simulink model "ICAC_AutoSave_20200630_1355"  (R2018b)
settings: Solver=FixedStepDiscrete  StartTime=0.0  StopTime=10.0  RelTol=1e-3
InitFcn:
  | tmpVer = ver('MATLAB');
  | tmpVer = str2num(tmpVer.Version);
  | % -------------------------------------------------------------------
  | %  MATLAB file generated by Simulink.saveVars on 21-Nov-2019 10:06:14
  | %  MATLAB version: 7.13.0.564 (R2011b)
  | % -------------------------------------------------------------------
  | 
  | 
  | SInt16 = Simulink.AliasType;
  | SInt16.Description = 'Num';
  | if (tmpVer > 7.11)
  | 	SInt16.DataScope = 'Auto';
  | end
  | SInt16.HeaderFile = 'Rte_Type.h';
  | SInt16.BaseType = 'int16';
  | 
  | SInt32 = Simulink.AliasType;
  | SInt32.Description = 'Num';
  | if (tmpVer > 7.11)
  | 	SInt32.DataScope = 'Auto';
  | end
  | SInt32.HeaderFile = 'Rte_Type.h';
  | SInt32.BaseType = 'int32';
  | 
  | SInt8 = Simulink.AliasType;
  | SInt8.Description = 'Num';
  | if (tmpVer > 7.11)
  | 	SInt8.DataScope = 'Auto';
  | end
  | SInt8.HeaderFile = 'Rte_Type.h';
  | SInt8.BaseType = 'int8';
  | 
  | T_A_m2_1024_1_u32 = Simulink.NumericType;
  | T_A_m2_1024_1_u32.Description = 'm2 (square meters  (m2))';
  | if (tmpVer > 7.11)
  | 	T_A_m2_1024_1_u32.DataScope = 'Auto';
  | end
  | T_A_m2_1024_1_u32.HeaderFile = 'Rte_Type.h';
  | T_A_m2_1024_1_u32.DataTypeMode = 'Fixed-point: slope and bias scaling';
  | T_A_m2_1024_1_u32.SignednessBool = false;
  | T_A_m2_1024_1_u32.WordLength = 32;
  | T_A_m2_1024_1_u32.FixedExponent = -10;
  | T_A_m2_1024_1_u32.SlopeAdjustmentFactor = 1;
  | T_A_m2_1024_1_u32.Bias = 0;
  | T_A_m2_1024_1_u32.DataTypeOverride = 'Inherit';
  | T_A_m2_1024_1_u32.IsAlias = true;
  | 
  | T_A_m2_65536_1_u16 = Simulink.NumericType;
  | T_A_m2_65536_1_u16.Description = 'm2 (square meters  (m2))';
  | if (tmpVer > 7.11)
  | 	T_A_m2_65536_1_u16.DataScope = 'Auto';
  | end
  | T_A_m2_65536_1_u16.HeaderFile = 'Rte_Type.h';
  | T_A_m2_65536_1_u16.DataTypeMode = 'Fixed-point: slope and bias scaling';
  | T_A_m2_65536_1_u16.SignednessBool = false;
  | T_A_m2_65536_1_u16.WordLength = 16;
  | T_A_m2_65536_1_u16.FixedExponent = -16;
  | T_A_m2_65536_1_u16.SlopeAdjustmentFactor = 1;
  | T_A_m2_65536_1_u16.Bias = 0;
  | T_A_m2_65536_1_u16.DataTypeOverride = 'Inherit';
  | ... (+4598 lines)
StopFcn:
  | clear  T_A_m2_1024_1_u32 T_A_m2_65536_1_u16 T_A_m2_Float32 T_A_mm2_10_1_u16 T_A_mm2_4_1_s16 T_A_mm2_Float32 T_Cnt_Num_10_1_u32 T_Cnt_Num_1_1_s16 T_Cnt_Num_1_1_s32 T_Cnt_Num_1_1_s8 T_Cnt_Num_1_1_u16 T_Cnt_Num_1_1_u32 T_Cnt_Num_1_1_u8 T_E_J_1_1_s32 T_E_J_Float32 T_E_kJ_128_1_s32 T_E_kJ_Float32 T_E_kwh_10_1_u16 T_E_kwh_Float32 T_Epl_kwhpkm_100_1_u16 T_Epl_kwhpkm_Float32 T_F_N_1_1_s16 T_F_N_Float32 T_I_A_1000_1_u16 T_I_A_1048576_1_s32 T_I_A_2048_1_s16 T_I_A_32_1_s16 T_I_A_Float32 T_I_mA_1_1_s16 T_I_mA_32768_128_s16 T_I_mA_Float32 T_J_kgpm2_128_1_u16 T_J_kgpm2_Float32 T_K_NA_1000_1_s16 T_K_NA_100_1_s16 T_K_NA_100_1_u16 T_K_NA_1024_1_s16 T_K_NA_1024_1_u16 T_K_NA_128_1_s16 T_K_NA_128_1_u16 T_K_NA_128_1_u8 T_K_NA_16777216_1_u32 T_K_NA_16_1_s16 T_K_NA_16_1_u16 T_K_NA_16_1_u8 T_K_NA_1_16_u16 T_K_NA_1_1_s16 T_K_NA_1_1_u16 T_K_NA_1_1_u8 T_K_NA_32768_1_s16 T_K_NA_32768_1_u16 T_K_NA_32_1_s8 T_K_NA_4096_1_u16 T_K_NA_4194304_1_s32 T_K_NA_4194304_1_u16 T_K_NA_65536_1_s32 T_K_NA_65536_1_u16 T_K_NA_8192_1_s16 T_K_NA_8_1_s16 T_K_NA_Float32 T_M_Nm_16_1_s16 T_M_Nm_1_1_s16 T_M_Nm_32768_1_s16 T_M_Nm_32_1_s16 T_M_Nm_4_1_s16 T_M_Nm_512_1_s16 T_M_Nm_Float32 T_P_W_1_4_s16 T_P_W_1_8_s16 T_P_W_Float32 T_P_kW_128_1_s16 T_P_kW_1_8_s16 T_P_kW_8_1_s32 T_P_kW_Float32 T_Pct_pct_1024_1_s32 T_Pct_pct_1024_1_u32 T_Pct_pct_10_1_s16 T_Pct_pct_10_1_u32 T_Pct_pct_128_100_s8 T_Pct_pct_1_1_s16 T_Pct_pct_1_4_u8 T_Pct_pct_255_100_u16 T_Pct_pct_255_100_u8 T_Pct_pct_256_1_s16 T_Pct_pct_256_1_u16 T_Pct_pct_65535_100_u16 T_Pct_pct_Float32 T_R_ohm_1024_1_s16 T_R_ohm_32_1_s16 T_R_ohm_Float32 T_TK_K_16_1_s16 T_TK_K_Float32 T_T_degC_10_400_1_u16 T_T_degC_16_1_s16 T_T_degC_1_40_1_u8 T_T_degC_2_80_1_u8 T_T_degC_Float32 T_U_V_1000_1_u16 T_U_V_10_1_u8 T_U_V_200_1_u8 T_U_V_32_1_s16 T_U_V_4096_1_s16 T_U_V_512_1_s16 T_U_V_65535_8_u16 T_U_V_8192_1_u16 T_U_V_Float32 T_U_mV_1_1_s16 T_U_mV_256_20_u16 T_U_mV_Float32 T_V_l_256_1_s16 T_V_l_4096_1_s16 T_V_l_64_1_s16 T_V_l_65535_100_u16 T_V_l_Float32 T_V_ml_128_1_s16 T_V_ml_1_1_s16 T_V_ml_32768_1_s16 T_V_ml_Float32 T_V_ul_32_1_u16 T_V_ul_Float32 T_Vpl_clpkm_512_1_u16 T_Vpl_clpkm_Float32 T_a_kphps_16_1_s16 T_a_kphps_Float32 T_a_mps2_128_1_s16 T_a_mps2_Float32 T_c_MJpkg_256_1_s16 T_c_MJpkg_Float32 T_c_kJpgpK_1024_1_s16 T_c_kJpgpK_Float32 T_c_kJpkgpK_128_1_u16 T_c_kJpkgpK_Float32 T_chrg_Ah_1_1_s16 T_chrg_Ah_1_1_u16 T_chrg_Ah_1_1_u8 T_chrg_Ah_256_1_u16 T_chrg_Ah_4194304_1_s32 T_chrg_Ah_512_1_u16 T_chrg_Ah_8_1_u16 T_chrg_Ah_Float32 T_cmp_NA_100_1_s16 T_cmp_NA_128_1_s16 T_cmp_NA_16_1_s16 T_cmp_NA_32768_1_u16 T_cmp_NA_Float32 T_d2n_rpmps2_4_1_s16 T_d2n_rpmps2_Float32 T_dPct_pctps_16_1_s16 T_dPct_pctps_256_1_s16 T_dPct_pctps_Float32 T_dT_degCps_128_1_s16 T_dT_degCps_Float32 T_dV_lph_1_1_s16 T_dV_lph_Float32 T_dV_lpm_128_1_s16 T_dV_lpm_32_1_s16 T_dV_lpm_Float32 T_dV_lps_1024_1_u16 T_dV_lps_4_1_u16 T_dV_lps_Float32 T_dV_mlps_1024_1_s16 T_dV_mlps_Float32 T_d_BitField16 T_dm_gps_128_1_s16 T_dm_gps_128_1_u16 T_dm_gps_256_1_u16 T_dm_gps_Float32 T_dm_mgps_1_1_s16 T_dm_mgps_Float32 T_dn_rpmps_1_1_s16 T_dn_rpmps_2_1_s16 T_dn_rpmps_Float32 T_dp_Paps_1_1_s16 T_dp_Paps_Float32 T_dp_kPaps_1_1_s16 T_dp_kPaps_8_1_s16 T_dp_kPaps_Float32 T_dphi_degps_128_1_s16 T_dphi_degps_8_1_s16 T_dphi_degps_Float32 T_dr_ps_256_1_s16 T_dr_ps_Float32 T_drho_mgplps_1_2_s16 T_drho_mgplps_Float32 T_e_NA_1_1_u8 T_f_Hz_1_1_u16 T_f_Hz_1_1_u32 T_f_Hz_64_1_u16 T_f_Hz_8_1_s16 T_f_Hz_Float32 T_g_BitField32 T_l_km_16_1_s16 T_l_km_1_1_u16 T_l_km_1_1_u32 T_l_km_Float32 T_l_m_1024_1_s16 T_l_m_16_1_s16 T_l_m_1_1_u32 T_l_m_Float32 T_l_mm_16_1_s16 T_l_mm_1_1_u16 T_l_mm_4096_1_s16 T_l_mm_4_1_u8 T_l_mm_64_1_s16 T_l_mm_Float32 T_m_g_1_1_s16 T_m_g_2048_1_s16 T_m_g_32_1_u16 T_m_g_Float32 T_m_kg_1024_1_s16 T_m_kg_1_1_s16 T_m_kg_1_1_u32 T_m_kg_Float32 T_m_mg_128_1_s16 T_m_mg_32_1_s16 T_m_mg_Float32 T_n_rpm_1_1_s16 T_n_rpm_1_25_u8 T_n_rpm_256_50_u16 T_n_rpm_2_25_u8 T_n_rpm_4_1_u16 T_n_rpm_Float32 T_p_MPa_64_1_s16 T_p_MPa_Float32 T_p_Pa_1_1_s16 T_p_Pa_Float32 T_p_kPa_1_10_u16 T_p_kPa_1_1_s16 T_p_kPa_1_1_u8 T_p_kPa_256_1_u16 T_p_kPa_32_1_u16 T_p_kPa_64_1_s16 T_p_kPa_Float32 T_phi_deg_100_1_s16 T_phi_deg_1024_1_s16 T_phi_deg_128_1_s16 T_phi_deg_1_1_u8 T_phi_deg_256_1_s16 T_phi_deg_2_1_s8 T_phi_deg_32_1_s16 T_phi_deg_512_6_s32 T_phi_deg_Float32 T_phi_rad_2048_1_s16 T_phi_rad_Float32 T_r_NA_1024_1_s16 T_r_NA_1024_1_u16 T_r_NA_16384_1_s16 T_r_NA_16_1_s16 T_r_NA_256_1_s8 T_r_NA_256_1_u16 T_r_NA_32768_1_u16 T_r_NA_32_1_u16 T_r_NA_4096_1_s16 T_r_NA_65535_2_u16 T_r_NA_8192_1_u16 T_r_NA_Float32 T_rho_gpl_8192_1_s16 T_rho_gpl_Float32 T_rho_kgpm3_16_1_s16 T_rho_kgpm3_Float32 T_rho_mgpl_1_1_s16 T_rho_mgpl_64_1_s16 T_rho_mgpl_Float32 T_t_hour_1_1_s16 T_t_hour_Float32 T_t_m_1_1_u16 T_t_m_Float32 T_t_ms_1_1_s16 T_t_ms_1_1_u16 T_t_ms_1_1_u32 T_t_ms_4096_1_s16 T_t_ms_64_1_s16 T_t_ms_Float32 T_t_s_1000_1_s16 T_t_s_100_1_s16 T_t_s_10_1_s16 T_t_s_10_1_u16 T_t_s_1_1_s16 T_t_s_1_1_u16 T_t_s_1_1_u32 T_t_s_Float32 T_t_us_10_1_u32 T_t_us_1_1_s16 T_t_us_1_1_u32 T_t_us_1_4_u16 T_t_us_Float32 T_v_kph_1_1_u8 T_v_kph_64_1_s16 T_v_kph_64_1_u16 T_v_kph_Float32 T_v_mps_256_1_s16 T_v_mps_Float32 T_w_radps_32_1_s16 T_w_radps_Float32 T_y_BitField8 T_y_BitFieldDiagProgress T_y_BitFieldDiagStatus T_y_NA_1_1_u8 SInt16 SInt32 SInt8 T_BOOLEAN UInt16 UInt32 UInt8 s16 s32 s8 u16 u32 u8
(part 3 of 3)

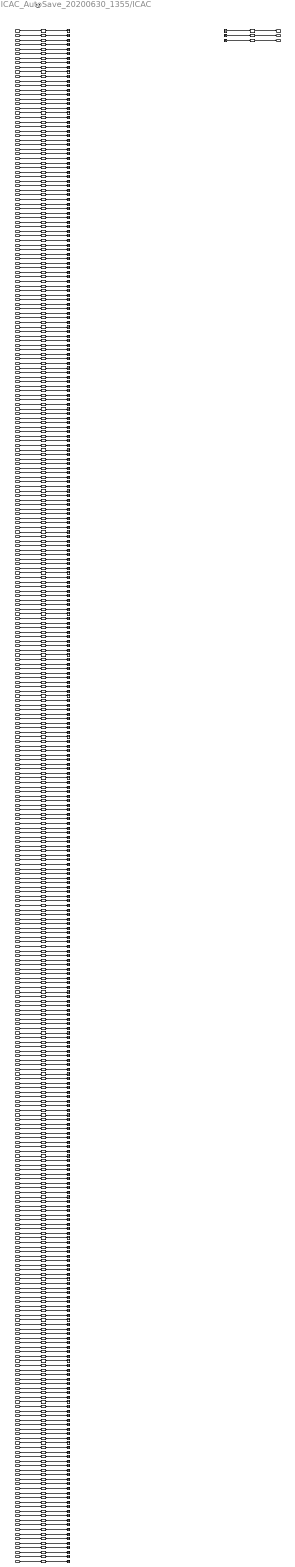
== system ICAC_AutoSave_20200630_1355/ICAC ==
  System_Clock : Inport
  ICABva_g_VehParameter : Inport  Port=2
  ICABva_g_FilterInfo : Inport  Port=3
  ICABve_d_SignalTStamp : Inport  Port=4
  ICAPva_g_PathPoints : Inport  Port=5
  ICAPve_d_PathPointNum : Inport  Port=6
  ICAPve_d_PathValid : Inport  Port=7
  ICAPve_d_SignalTStamp : Inport  Port=8
  ICASva_g_TrajectoryPoints : Inport  Port=9
  ICASve_d_TrajectoryPointNum : Inport  Port=10
  ICASve_d_TrajectoryValid : Inport  Port=11
  ICASva_d_TrajectoryPlanState : Inport  Port=12
  ICASve_g_ExpLonAcc : Inport  Port=13
  ICASve_d_SignalTStamp : Inport  Port=14
  IMAPve_d_EPS_LKA_State : Inport  Port=15
  IMAPve_g_EPS_SW_Trq : Inport  Port=16
  IMAPve_d_EPS_Error_State : Inport  Port=17
  IMAPve_d_EPS_Trq_State : Inport  Port=18
  IMAPve_d_SAS_Clb_State : Inport  Port=19
  IMAPve_d_SAS_Trim_State : Inport  Port=20
  IMAPve_d_EPS_TrqLim_State : Inport  Port=21
  IMAPve_g_EPS_LKA_Current : Inport  Port=22
  IMAPve_g_ESC_LatAcc : Inport  Port=23
  IMAPve_d_ESC_LatAcc_Valid : Inport  Port=24
  IMAPve_g_ESC_YawRate : Inport  Port=25
  IMAPve_d_ESC_YawRate_Valid : Inport  Port=26
  IMAPve_g_ESC_UnYawRate : Inport  Port=27
  IMAPve_g_ESC_VehSpd : Inport  Port=28
  IMAPve_g_ESC_LonAcc : Inport  Port=29
  IMAPve_d_ESC_LonAcc_Valid : Inport  Port=30
  IMAPve_g_ESC_Brake_Press : Inport  Port=31
  IMAPve_g_ESC_Static_Slope : Inport  Port=32
  IMAPve_g_ESC_DySlope_Accuracy : Inport  Port=33
  IMAPve_g_ESC_DySlope : Inport  Port=34
  IMAPve_g_SW_Angle : Inport  Port=35
  IMAPve_g_SW_Angle_Speed : Inport  Port=36
  IMAPve_d_BCM_HazardLamp : Inport  Port=37
  IMAPve_d_BCM_Left_Light : Inport  Port=38
  IMAPve_d_BCM_Right_Light : Inport  Port=39
  IMAPve_d_ESC_BrakeLamp_Req : Inport  Port=40
  IMAPve_d_BCM_Opening_State : Inport  Port=41
  IMAPve_d_BCM_Trunk_State : Inport  Port=42
  IMAPve_d_BCM_LF_Door_State : Inport  Port=43
  IMAPve_d_BCM_RF_Door_State : Inport  Port=44
  IMAPve_d_BCM_RR_Door_State : Inport  Port=45
  IMAPve_d_BCM_LR_Door_State : Inport  Port=46
  IMAPve_d_SCC_Left_SwitchSig : Inport  Port=47
  IMAPve_d_SCC_Right_SwitchSig : Inport  Port=48
  IMAPve_d_PEPS_Door_Lock_Req : Inport  Port=49
  IMAPve_d_BCM_Door_Lock_State : Inport  Port=50
  IMAPve_d_EMS_ACC_Status : Inport  Port=51
  IMAPve_g_EMS_Pot_WhlT_Max : Inport  Port=52
  IMAPve_g_EMS_Pot_WhlT_Min : Inport  Port=53
  IMAPve_g_EMS_RealPedal : Inport  Port=54
  IMAPve_g_EMS_MaxTWhl : Inport  Port=55
  IMAPve_g_EMS_MaxTWhl_Offset : Inport  Port=56
  IMAPve_g_EMS_MinTWhl : Inport  Port=57
  IMAPve_g_EMS_MinTWhl_Offset : Inport  Port=58
  IMAPve_g_EMS_Actual_FlwT : Inport  Port=59
  IMAPve_g_EMS_Actual_IndT : Inport  Port=60
  IMAPve_g_EMS_Realize_TWhl : Inport  Port=61
  IMAPve_g_EMS_ACC_VirtualPedal : Inport  Port=62
  IMAPve_d_EMS_AccPedal_Fault : Inport  Port=63
  IMAPve_g_EMS_Driver_Torque : Inport  Port=64
  IMAPve_d_ESC_Brake_Effort : Inport  Port=65
  IMAPve_g_EMS_Engine_Speed : Inport  Port=66
  IMAPve_d_ESC_Veh_Standstill : Inport  Port=67
  IMAPve_d_TCU_Actual_Gear : Inport  Port=68
  IMAPve_d_TCU_Target_Gear : Inport  Port=69
  IMAPve_d_TCU_PRND_State : Inport  Port=70
  IMAPve_d_BCM_Ignition_State : Inport  Port=71
  IMAPve_d_ACU_Driver_Belt : Inport  Port=72
  IMAPve_d_SWS_Fault_Code : Inport  Port=73
  IMAPve_d_SWS_Failure_Status : Inport  Port=74
  IMAPve_d_ESC_OFF : Inport  Port=75
  IMAPve_d_ESC_AlarmSig : Inport  Port=76
  IMAPve_d_Speed_Limit_Switch : Inport  Port=77
  IMAPve_d_ESC_ESC_Active : Inport  Port=78
  IMAPve_d_ESC_MSR_Active : Inport  Port=79
  IMAPve_d_ESC_TCS_Active : Inport  Port=80
  IMAPve_d_ESC_VehSpd_Valid : Inport  Port=81
  IMAPve_d_Brake_Pedal_Fault : Inport  Port=82
  IMAPve_d_ESC_ABS_Active : Inport  Port=83
  IMAPve_d_ESC_ABS_Valid : Inport  Port=84
  IMAPve_d_ESC_ABS_AlarmSig : Inport  Port=85
  IMAPve_d_ESC_FL_WheelPulVal : Inport  Port=86
  IMAPve_d_ESC_FR_WheelPulVal : Inport  Port=87
  IMAPve_d_ESC_RL_WheelPulVal : Inport  Port=88
  IMAPve_d_ESC_RR_WheelPulVal : Inport  Port=89
  IMAPve_g_ESC_FL_WhlSpd : Inport  Port=90
  IMAPve_d_ESC_FL_WhlSpd_Fault : Inport  Port=91
  IMAPve_g_ESC_FR_WhlSpd : Inport  Port=92
  IMAPve_d_ESC_FR_WhlSpd_Fault : Inport  Port=93
  IMAPve_g_ESC_RL_WhlSpd : Inport  Port=94
  IMAPve_d_ESC_RL_WhlSpd_Fault : Inport  Port=95
  IMAPve_g_ESC_RR_WhlSpd : Inport  Port=96
  IMAPve_d_ESC_RR_WhlSpd_Fault : Inport  Port=97
  IMAPve_d_ESC_FL_Wheel_Pulse : Inport  Port=98
  IMAPve_d_ESC_FR_Wheel_Pulse : Inport  Port=99
  IMAPve_d_ESC_RL_Wheel_Pulse : Inport  Port=100
  IMAPve_d_ESC_RR_Wheel_Pulse : Inport  Port=101
  IMAPve_d_TCU_AT_Failure : Inport  Port=102
  IMAPve_d_TCU_Shift_Valid : Inport  Port=103
  IMAPve_d_TCU_DCT_Clutch_State : Inport  Port=104
  IMAPve_d_TCU_Gear_Engage : Inport  Port=105
  IMAPve_d_TCU_Select_ATMode : Inport  Port=106
  IMAPve_d_EMS_Engine_Status : Inport  Port=107
  IMAPve_d_EMS_Gearbox_CtlAvail : Inport  Port=108
  IMAPve_d_ESC_Brake_Failsafe : Inport  Port=109
  IMAPve_d_ESC_AEB_Status : Inport  Port=110
  IMAPve_d_ESC_AEB_Available : Inport  Port=111
  IMAPve_d_ESC_AEB_Active : Inport  Port=112
  IMAPve_d_ESC_ACC_Status : Inport  Port=113
  IMAPve_d_ESC_ACC_Available : Inport  Port=114
  IMAPve_d_ESC_ACC_Active : Inport  Port=115
  IMAPve_d_EMS_ACC_Effective : Inport  Port=116
  IMAPve_d_BCM_FrontWiper_State : Inport  Port=117
  IMAPve_d_BCM_CHMSL_Status : Inport  Port=118
  IMAPve_d_BCM_BrakeLamp_State : Inport  Port=119
  IMAPve_d_GW_Brake_Only_Req : Inport  Port=120
  IMAPve_d_ACU_Passenger_Belt : Inport  Port=121
  IMAPve_d_EMS_ACC_CtlAvail : Inport  Port=122
  IMAPve_d_EMS_ACC_Inhibited : Inport  Port=123
  IMAPve_d_EMS_Brake_Pedal : Inport  Port=124
  IMAPve_d_BCM_LowBeam_State : Inport  Port=125
  IMAPve_d_BCM_HighBeam_State : Inport  Port=126
  IMAPve_d_EPB_Status : Inport  Port=127
  IMAPve_d_EPB_Display_Req : Inport  Port=128
  IMAPve_d_EPB_Warn_Req : Inport  Port=129
  IMAPve_d_EPB_Switch_State : Inport  Port=130
  IMAPve_d_EPB_Switch_Valid : Inport  Port=131
  IMAPve_d_ESC_Drive_Direction : Inport  Port=132
  IMAPve_d_ESC_Hold_State : Inport  Port=133
  IMAPve_d_EPS_Steer_Hold_State : Inport  Port=134
  IMAPve_d_EPS_Warning_State : Inport  Port=135
  IMAPve_g_EPS_PowerCon : Inport  Port=136
  IMAPve_d_ESC_EBD_AlarmSig : Inport  Port=137
  IMAPve_d_ESC_AVH_Status : Inport  Port=138
  IMAPve_d_Radar_Detective_Req : Inport  Port=139
  IMAPve_g_BCM_Battery_Voltage : Inport  Port=140
  IMAPve_d_TBOX_LocalTimeY : Inport  Port=141
  IMAPve_d_TBOX_LocalTimeM : Inport  Port=142
  IMAPve_d_TBOX_LocalTimeD : Inport  Port=143
  IMAPve_d_TBOX_LocalTimeH : Inport  Port=144
  IMAPve_d_TBOX_LocalTimeMin : Inport  Port=145
  IMAPve_d_TBOX_LocalTimeS : Inport  Port=146
  IMAPve_d_TBOX_LocalTime_Valid : Inport  Port=147
  IMAPve_d_TPMS_Warn_Indicate : Inport  Port=148
  IMAPve_d_Radar_State : Inport  Port=149
  IMAPve_d_ACC_Desired_Headway : Inport  Port=150
  IMAPve_d_Time_System_Clock : Inport  Port=151
  IMAPve_d_Signal_Time_Stamp : Inport  Port=152
  IMAPve_g_GW_IC_Odometer : Inport  Port=153
  IMAPve_g_FAPA_State : Inport  Port=154
  IMAPve_d_Outside_Temp : Inport  Port=155
  IMAPve_d_ORI_CIPV_ID : Inport  Port=156
  IMAPve_d_ORI_Obj_Num : Inport  Port=157
  IMAPva_g_ORI_Probability : Inport  Port=158
  IMAPva_d_ORI_Obj_Class : Inport  Port=159
  IMAPva_d_ORI_Obj_Motion : Inport  Port=160
  IMAPva_g_ORI_Obj_RelVel : Inport  Port=161
  IMAPva_g_ORI_Obj_LongDis : Inport  Port=162
  IMAPva_d_ORI_Obj_Lane : Inport  Port=163
  IMAPva_g_ORI_Obj_LAngle : Inport  Port=164
  IMAPva_g_ORI_Obj_RAngle : Inport  Port=165
  IMAPva_g_ORI_Obj_Width : Inport  Port=166
  IMAPva_d_ORI_Obj_ID : Inport  Port=167
  IMAPve_d_ORI_Lane_Valid : Inport  Port=168
  IMAPve_d_ORI_Lane_ConsArea : Inport  Port=169
  IMAPve_d_ORI_Lane_RoadType : Inport  Port=170
  IMAPve_g_ORI_L0_C3 : Inport  Port=171
  IMAPve_g_ORI_L0_C2 : Inport  Port=172
  IMAPve_g_ORI_L0_C1 : Inport  Port=173
  IMAPve_g_ORI_L0_C0 : Inport  Port=174
  IMAPve_d_ORI_L0_Q : Inport  Port=175
  IMAPve_d_ORI_L0_Type : Inport  Port=176
  IMAPve_g_ORI_L0_VR : Inport  Port=177
  IMAPve_g_ORI_L0_TLC : Inport  Port=178
  IMAPve_g_ORI_L0_W : Inport  Port=179
  IMAPve_d_ORI_L0_LC : Inport  Port=180
  IMAPve_g_ORI_L1_C3 : Inport  Port=181
  IMAPve_g_ORI_L1_C2 : Inport  Port=182
  IMAPve_g_ORI_L1_C1 : Inport  Port=183
  IMAPve_g_ORI_L1_C0 : Inport  Port=184
  IMAPve_d_ORI_L1_Q : Inport  Port=185
  IMAPve_d_ORI_L1_Type : Inport  Port=186
  IMAPve_g_ORI_L1_VR : Inport  Port=187
  IMAPve_g_ORI_L1_TLC : Inport  Port=188
  IMAPve_g_ORI_L1_W : Inport  Port=189
  IMAPve_d_ORI_L1_LC : Inport  Port=190
  IMAPve_g_ORI_R0_C3 : Inport  Port=191
  IMAPve_g_ORI_R0_C2 : Inport  Port=192
  IMAPve_g_ORI_R0_C1 : Inport  Port=193
  IMAPve_g_ORI_R0_C0 : Inport  Port=194
  IMAPve_d_ORI_R0_Q : Inport  Port=195
  IMAPve_d_ORI_R0_LT : Inport  Port=196
  IMAPve_g_ORI_R0_VR : Inport  Port=197
  IMAPve_g_ORI_R0_TLC : Inport  Port=198
  IMAPve_g_ORI_R0_W : Inport  Port=199
  IMAPve_d_ORI_R0_LC : Inport  Port=200
  IMAPve_g_ORI_R1_C3 : Inport  Port=201
  IMAPve_g_ORI_R1_C2 : Inport  Port=202
  IMAPve_g_ORI_R1_C1 : Inport  Port=203
  IMAPve_g_ORI_R1_C0 : Inport  Port=204
  IMAPve_d_ORI_R1_Q : Inport  Port=205
  IMAPve_d_ORI_R1_LT : Inport  Port=206
  IMAPve_g_ORI_R1_VR : Inport  Port=207
  IMAPve_g_ORI_R1_TLC : Inport  Port=208
  IMAPve_g_ORI_R1_W : Inport  Port=209
  IMAPve_d_ORI_R1_LC : Inport  Port=210
  IMAPve_d_Sensor_Status : Inport  Port=211
  IMAPve_d_LF_Radar_Status : Inport  Port=212
  IMAPve_d_RF_Radar_Status : Inport  Port=213
  IMAPve_d_LR_Radar_Status : Inport  Port=214
  IMAPve_d_RR_Radar_Status : Inport  Port=215
  IMAPve_d_Fusion_Status : Inport  Port=216
  IMAPve_g_Fusion_Time_Stamp : Inport  Port=217
  IMAPve_d_obj_Num : Inport  Port=218
  IMAPva_d_obj_id : Inport  Port=219
  IMAPva_g_obj_pos_x : Inport  Port=220
  IMAPva_g_obj_pos_y : Inport  Port=221
  IMAPva_g_obj_vel_x : Inport  Port=222
  IMAPva_g_obj_vel_y : Inport  Port=223
  IMAPva_g_obj_acc_x : Inport  Port=224
  IMAPva_g_obj_acc_y : Inport  Port=225
  IMAPva_g_obj_pos_var_x : Inport  Port=226
  IMAPva_g_obj_pos_var_y : Inport  Port=227
  IMAPva_g_obj_pos_var_xy : Inport  Port=228
  IMAPva_g_obj_vel_var_x : Inport  Port=229
  IMAPva_g_obj_vel_var_y : Inport  Port=230
  IMAPva_g_obj_vel_var_xy : Inport  Port=231
  IMAPva_g_obj_width : Inport  Port=232
  IMAPva_g_obj_length : Inport  Port=233
  IMAPva_d_obj_fusion_type : Inport  Port=234
  IMAPva_d_obj_class : Inport  Port=235
  IMAPva_d_obj_lane : Inport  Port=236
  IMAPva_d_obj_status : Inport  Port=237
  IMAPva_d_obj_cam_asso_id : Inport  Port=238
  IMAPva_g_obj_con : Inport  Port=239
  IMAPva_g_obj_age : Inport  Port=240
  IMAPva_d_obj_TurnLight : Inport  Port=241
  IMAPva_d_obj_BrakeLight : Inport  Port=242
  IMAPva_d_obj_MotionStatus : Inport  Port=243
  IMAPva_d_obj_ACC : Inport  Port=244
  IMAPva_d_obj_AEB : Inport  Port=245
  IMAPva_d_obj_ELK : Inport  Port=246
  IMAPva_d_obj_ALC : Inport  Port=247
  IMAPva_d_obj_ESA : Inport  Port=248
  IMAPva_d_obj_JA : Inport  Port=249
  IMAPve_d_Lane_Valid : Inport  Port=250
  IMAPve_d_Road_Type : Inport  Port=251
  IMAPve_d_ConsArea : Inport  Port=252
  IMAPve_g_L0_C0 : Inport  Port=253
  IMAPve_g_L0_C1 : Inport  Port=254
  IMAPve_g_L0_C2 : Inport  Port=255
  IMAPve_g_L0_C3 : Inport  Port=256
  IMAPve_g_L0_VR : Inport  Port=257
  IMAPve_d_L0_Q : Inport  Port=258
  IMAPve_d_L0_Type : Inport  Port=259
  IMAPve_g_L0_Confidence : Inport  Port=260
  IMAPve_g_L0_W : Inport  Port=261
  IMAPve_g_L0_TLC : Inport  Port=262
  IMAPve_d_L0_LC : Inport  Port=263
  IMAPve_g_R0_C0 : Inport  Port=264
  IMAPve_g_R0_C1 : Inport  Port=265
  IMAPve_g_R0_C2 : Inport  Port=266
  IMAPve_g_R0_C3 : Inport  Port=267
  IMAPve_g_R0_VR : Inport  Port=268
  IMAPve_d_R0_Q : Inport  Port=269
  IMAPve_d_R0_Type : Inport  Port=270
  IMAPve_g_R0_Confidence : Inport  Port=271
  IMAPve_g_R0_W : Inport  Port=272
  IMAPve_g_R0_TLC : Inport  Port=273
  IMAPve_d_R0_LC : Inport  Port=274
  IMAPve_g_L1_C0 : Inport  Port=275
  IMAPve_g_L1_C1 : Inport  Port=276
  IMAPve_g_L1_C2 : Inport  Port=277
  IMAPve_g_L1_C3 : Inport  Port=278
  IMAPve_g_L1_VR : Inport  Port=279
  IMAPve_d_L1_Q : Inport  Port=280
  IMAPve_d_L1_Type : Inport  Port=281
  IMAPve_g_L1_Confidence : Inport  Port=282
  IMAPve_g_L1_W : Inport  Port=283
  IMAPve_g_L1_TLC : Inport  Port=284
  IMAPve_d_L1_LC : Inport  Port=285
  IMAPve_g_R1_C0 : Inport  Port=286
  IMAPve_g_R1_C1 : Inport  Port=287
  IMAPve_g_R1_C2 : Inport  Port=288
  IMAPve_g_R1_C3 : Inport  Port=289
  IMAPve_g_R1_VR : Inport  Port=290
  IMAPve_d_R1_Q : Inport  Port=291
  IMAPve_d_R1_Type : Inport  Port=292
  IMAPve_g_R1_Confidence : Inport  Port=293
  IMAPve_g_R1_W : Inport  Port=294
  IMAPve_g_R1_TLC : Inport  Port=295
  IMAPve_d_R1_LC : Inport  Port=296
  IMAPve_g_L0_C0_Back : Inport  Port=297
  IMAPve_g_L0_C1_Back : Inport  Port=298
  IMAPve_g_L0_C2_Back : Inport  Port=299
  IMAPve_g_L0_C3_Back : Inport  Port=300
  IMAPve_g_L0_Range_Back : Inport  Port=301
  IMAPve_g_L0_C0_FR_Pred : Inport  Port=302
  IMAPve_g_L0_C1_FR_Pred : Inport  Port=303
  IMAPve_g_L0_C2_FR_Pred : Inport  Port=304
  IMAPve_g_L0_Range_FR_Pred : Inport  Port=305
  IMAPve_g_R0_C0_Back : Inport  Port=306
  IMAPve_g_R0_C1_Back : Inport  Port=307
  IMAPve_g_R0_C2_Back : Inport  Port=308
  IMAPve_g_R0_C3_Back : Inport  Port=309
  IMAPve_g_R0_Range_Back : Inport  Port=310
  IMAPve_g_R0_C0_FR_Pred : Inport  Port=311
  IMAPve_g_R0_C1_FR_Pred : Inport  Port=312
  IMAPve_g_R0_C2_FR_Pred : Inport  Port=313
  IMAPve_g_R0_Range_FR_Pred : Inport  Port=314
  IMAPve_g_L1_C0_Back : Inport  Port=315
  IMAPve_g_L1_C1_Back : Inport  Port=316
  IMAPve_g_L1_C2_Back : Inport  Port=317
  IMAPve_g_L1_C3_Back : Inport  Port=318
  IMAPve_g_L1_Range_Back : Inport  Port=319
  IMAPve_g_L1_C0_FR_Pred : Inport  Port=320
  IMAPve_g_L1_C1_FR_Pred : Inport  Port=321
  IMAPve_g_L1_C2_FR_Pred : Inport  Port=322
  IMAPve_g_L1_Range_FR_Pred : Inport  Port=323
  IMAPve_g_R1_C0_Back : Inport  Port=324
  IMAPve_g_R1_C1_Back : Inport  Port=325
  IMAPve_g_R1_C2_Back : Inport  Port=326
  IMAPve_g_R1_C3_Back : Inport  Port=327
  IMAPve_g_R1_Range_Back : Inport  Port=328
  IMAPve_g_R1_C0_FR_Pred : Inport  Port=329
  IMAPve_g_R1_C1_FR_Pred : Inport  Port=330
  IMAPve_g_R1_C2_FR_Pred : Inport  Port=331
  IMAPve_g_R1_Range_FR_Pred : Inport  Port=332
  IMAPve_d_Sign_ISA_Value : Inport  Port=333
  IMAPve_d_TSR_Sign_Type : Inport  Port=334
  IMAPve_d_Camera_Signal_Fault : Inport  Port=335
  IMAPve_d_Radar_Status : Inport  Port=336
  IMAPve_d_Camera_Status : Inport  Port=337
  function : TriggerPort  TriggerType=function-call  VariantControl=Variant  SampleTimeType=periodic  SampleTime=-1
  ICABva_g_FilterInfo_1 : DataTypeConversion  OutDataTypeStr=single
  ICABva_g_FilterInfo_2 : Terminator
  ICABva_g_VehParameter1 : Terminator
  ICABva_g_VehParameter_1 : DataTypeConversion  OutDataTypeStr=single
  ICABve_d_SignalTStamp_1 : DataTypeConversion  OutDataTypeStr=uint16
  ICABve_d_SignalTStamp_2 : Terminator
  ICACve_d_SignalTStamp_1 : DataTypeConversion  OutDataTypeStr=UInt16
  ICACve_d_SignalTStamp_2 : Ground
  ICACve_d_SteerAngleVld_1 : DataTypeConversion  OutDataTypeStr=UInt16
  ICACve_d_SteerAngleVld_2 : Ground
  ICACve_g_SteerAngleCmd_1 : DataTypeConversion  OutDataTypeStr=T_M_Nm_Float32
  ICACve_g_SteerAngleCmd_2 : Ground
  ICAPva_g_PathPoints_1 : DataTypeConversion  OutDataTypeStr=single
  ICAPva_g_PathPoints_2 : Terminator
  ICAPve_d_PathPointNum_1 : DataTypeConversion  OutDataTypeStr=uint16
  ICAPve_d_PathPointNum_2 : Terminator
  ICAPve_d_PathValid_1 : DataTypeConversion  OutDataTypeStr=uint16
  ICAPve_d_PathValid_2 : Terminator
  ICAPve_d_SignalTStamp_1 : DataTypeConversion  OutDataTypeStr=uint16
  ICAPve_d_SignalTStamp_2 : Terminator
  ICASva_d_TrajectoryPlanState_1 : DataTypeConversion  OutDataTypeStr=uint16
  ICASva_d_TrajectoryPlanState_2 : Terminator
  ICASva_g_TrajectoryPoints_1 : DataTypeConversion  OutDataTypeStr=single
  ICASva_g_TrajectoryPoints_2 : Terminator
  ICASve_d_SignalTStamp_1 : DataTypeConversion  OutDataTypeStr=uint16
  ICASve_d_SignalTStamp_2 : Terminator
  ICASve_d_TrajectoryPointNum_1 : DataTypeConversion  OutDataTypeStr=uint16
  ICASve_d_TrajectoryPointNum_2 : Terminator
  ICASve_d_TrajectoryValid_1 : DataTypeConversion  OutDataTypeStr=uint16
  ICASve_d_TrajectoryValid_2 : Terminator
  ICASve_g_ExpLonAcc_1 : DataTypeConversion  OutDataTypeStr=single
  ICASve_g_ExpLonAcc_2 : Terminator
  IMAPva_d_ORI_Obj_Class_1 : DataTypeConversion  OutDataTypeStr=uint16
  IMAPva_d_ORI_Obj_Class_2 : Terminator
  IMAPva_d_ORI_Obj_ID_1 : DataTypeConversion  OutDataTypeStr=uint16
  IMAPva_d_ORI_Obj_ID_2 : Terminator
  IMAPva_d_ORI_Obj_Lane_1 : DataTypeConversion  OutDataTypeStr=uint16
  IMAPva_d_ORI_Obj_Lane_2 : Terminator
  IMAPva_d_ORI_Obj_Motion_1 : DataTypeConversion  OutDataTypeStr=uint16
  IMAPva_d_ORI_Obj_Motion_2 : Terminator
  IMAPva_d_obj_ACC_1 : DataTypeConversion  OutDataTypeStr=uint16
  IMAPva_d_obj_ACC_2 : Terminator
  IMAPva_d_obj_AEB_1 : DataTypeConversion  OutDataTypeStr=uint16
  IMAPva_d_obj_AEB_2 : Terminator
  IMAPva_d_obj_ALC_1 : DataTypeConversion  OutDataTypeStr=uint16
  IMAPva_d_obj_ALC_2 : Terminator
  IMAPva_d_obj_BrakeLight_1 : DataTypeConversion  OutDataTypeStr=uint16
  IMAPva_d_obj_BrakeLight_2 : Terminator
  IMAPva_d_obj_ELK_1 : DataTypeConversion  OutDataTypeStr=uint16
  IMAPva_d_obj_ELK_2 : Terminator
  IMAPva_d_obj_ESA_1 : DataTypeConversion  OutDataTypeStr=uint16
  IMAPva_d_obj_ESA_2 : Terminator
  IMAPva_d_obj_JA_1 : DataTypeConversion  OutDataTypeStr=uint16
  IMAPva_d_obj_JA_2 : Terminator
  IMAPva_d_obj_MotionStatus_1 : DataTypeConversion  OutDataTypeStr=uint16
  IMAPva_d_obj_MotionStatus_2 : Terminator
  IMAPva_d_obj_TurnLight_1 : DataTypeConversion  OutDataTypeStr=uint16
  IMAPva_d_obj_TurnLight_2 : Terminator
  IMAPva_d_obj_cam_asso_id_1 : DataTypeConversion  OutDataTypeStr=uint16
  IMAPva_d_obj_cam_asso_id_2 : Terminator
  IMAPva_d_obj_class_1 : DataTypeConversion  OutDataTypeStr=uint16
  IMAPva_d_obj_class_2 : Terminator
  IMAPva_d_obj_fusion_type_1 : DataTypeConversion  OutDataTypeStr=uint16
  IMAPva_d_obj_fusion_type_2 : Terminator
  IMAPva_d_obj_id_1 : DataTypeConversion  OutDataTypeStr=uint16
  IMAPva_d_obj_id_2 : Terminator
  IMAPva_d_obj_lane_1 : DataTypeConversion  OutDataTypeStr=uint16
  IMAPva_d_obj_lane_2 : Terminator
  IMAPva_d_obj_status_1 : DataTypeConversion  OutDataTypeStr=uint16
  IMAPva_d_obj_status_2 : Terminator
  IMAPva_g_ORI_Obj_LAngle_1 : DataTypeConversion  OutDataTypeStr=single
  IMAPva_g_ORI_Obj_LAngle_2 : Terminator
  IMAPva_g_ORI_Obj_LongDis_1 : DataTypeConversion  OutDataTypeStr=single
  IMAPva_g_ORI_Obj_LongDis_2 : Terminator
  IMAPva_g_ORI_Obj_RAngle_1 : DataTypeConversion  OutDataTypeStr=single
  IMAPva_g_ORI_Obj_RAngle_2 : Terminator
  IMAPva_g_ORI_Obj_RelVel_1 : DataTypeConversion  OutDataTypeStr=single
  IMAPva_g_ORI_Obj_RelVel_2 : Terminator
  IMAPva_g_ORI_Obj_Width_1 : DataTypeConversion  OutDataTypeStr=single
  IMAPva_g_ORI_Obj_Width_2 : Terminator
  IMAPva_g_ORI_Probability_1 : DataTypeConversion  OutDataTypeStr=single
  IMAPva_g_ORI_Probability_2 : Terminator
  IMAPva_g_obj_acc_x_1 : DataTypeConversion  OutDataTypeStr=single
  IMAPva_g_obj_acc_x_2 : Terminator
  IMAPva_g_obj_acc_y_1 : DataTypeConversion  OutDataTypeStr=single
  IMAPva_g_obj_acc_y_2 : Terminator
  IMAPva_g_obj_age_1 : DataTypeConversion  OutDataTypeStr=single
  IMAPva_g_obj_age_2 : Terminator
  IMAPva_g_obj_con_1 : DataTypeConversion  OutDataTypeStr=single
  IMAPva_g_obj_con_2 : Terminator
  IMAPva_g_obj_length_1 : DataTypeConversion  OutDataTypeStr=single
  IMAPva_g_obj_length_2 : Terminator
  IMAPva_g_obj_pos_var_x_1 : DataTypeConversion  OutDataTypeStr=single
  IMAPva_g_obj_pos_var_x_2 : Terminator
  IMAPva_g_obj_pos_var_xy_1 : DataTypeConversion  OutDataTypeStr=single
  IMAPva_g_obj_pos_var_xy_2 : Terminator
  IMAPva_g_obj_pos_var_y_1 : DataTypeConversion  OutDataTypeStr=single
  IMAPva_g_obj_pos_var_y_2 : Terminator
  IMAPva_g_obj_pos_x_1 : DataTypeConversion  OutDataTypeStr=single
  IMAPva_g_obj_pos_x_2 : Terminator
  IMAPva_g_obj_pos_y_1 : DataTypeConversion  OutDataTypeStr=single
  IMAPva_g_obj_pos_y_2 : Terminator
  IMAPva_g_obj_vel_var_x_1 : DataTypeConversion  OutDataTypeStr=single
  IMAPva_g_obj_vel_var_x_2 : Terminator
  IMAPva_g_obj_vel_var_xy_1 : DataTypeConversion  OutDataTypeStr=single
  IMAPva_g_obj_vel_var_xy_2 : Terminator
  IMAPva_g_obj_vel_var_y_1 : DataTypeConversion  OutDataTypeStr=single
  IMAPva_g_obj_vel_var_y_2 : Terminator
  IMAPva_g_obj_vel_x_1 : DataTypeConversion  OutDataTypeStr=single
  IMAPva_g_obj_vel_x_2 : Terminator
  IMAPva_g_obj_vel_y_1 : DataTypeConversion  OutDataTypeStr=single
  IMAPva_g_obj_vel_y_2 : Terminator
  IMAPva_g_obj_width_1 : DataTypeConversion  OutDataTypeStr=single
  IMAPva_g_obj_width_2 : Terminator
  IMAPve_d_ACC_Desired_Headway_1 : DataTypeConversion  OutDataTypeStr=uint16
  IMAPve_d_ACC_Desired_Headway_2 : Terminator
  IMAPve_d_ACU_Driver_Belt_1 : DataTypeConversion  OutDataTypeStr=uint16
  IMAPve_d_ACU_Driver_Belt_2 : Terminator
  IMAPve_d_ACU_Passenger_Belt_1 : DataTypeConversion  OutDataTypeStr=uint16
  IMAPve_d_ACU_Passenger_Belt_2 : Terminator
  IMAPve_d_BCM_BrakeLamp_State_1 : DataTypeConversion  OutDataTypeStr=uint16
  IMAPve_d_BCM_BrakeLamp_State_2 : Terminator
  IMAPve_d_BCM_CHMSL_Status_1 : DataTypeConversion  OutDataTypeStr=uint16
  IMAPve_d_BCM_CHMSL_Status_2 : Terminator
  IMAPve_d_BCM_Door_Lock_State_1 : DataTypeConversion  OutDataTypeStr=uint16
  IMAPve_d_BCM_Door_Lock_State_2 : Terminator
  IMAPve_d_BCM_FrontWiper_State_1 : DataTypeConversion  OutDataTypeStr=uint16
  IMAPve_d_BCM_FrontWiper_State_2 : Terminator
  IMAPve_d_BCM_HazardLamp_1 : DataTypeConversion  OutDataTypeStr=uint16
  IMAPve_d_BCM_HazardLamp_2 : Terminator
  IMAPve_d_BCM_HighBeam_State_1 : DataTypeConversion  OutDataTypeStr=uint16
  IMAPve_d_BCM_HighBeam_State_2 : Terminator
  IMAPve_d_BCM_Ignition_State_1 : DataTypeConversion  OutDataTypeStr=uint16
  IMAPve_d_BCM_Ignition_State_2 : Terminator
  IMAPve_d_BCM_LF_Door_State_1 : DataTypeConversion  OutDataTypeStr=uint16
  IMAPve_d_BCM_LF_Door_State_2 : Terminator
  IMAPve_d_BCM_LR_Door_State_1 : DataTypeConversion  OutDataTypeStr=uint16
  IMAPve_d_BCM_LR_Door_State_2 : Terminator
  IMAPve_d_BCM_Left_Light_1 : DataTypeConversion  OutDataTypeStr=uint16
  IMAPve_d_BCM_Left_Light_2 : Terminator
  IMAPve_d_BCM_LowBeam_State_1 : DataTypeConversion  OutDataTypeStr=uint16
  IMAPve_d_BCM_LowBeam_State_2 : Terminator
  IMAPve_d_BCM_Opening_State_1 : DataTypeConversion  OutDataTypeStr=uint16
  IMAPve_d_BCM_Opening_State_2 : Terminator
  IMAPve_d_BCM_RF_Door_State_1 : DataTypeConversion  OutDataTypeStr=uint16
  IMAPve_d_BCM_RF_Door_State_2 : Terminator
  IMAPve_d_BCM_RR_Door_State_1 : DataTypeConversion  OutDataTypeStr=uint16
  IMAPve_d_BCM_RR_Door_State_2 : Terminator
  IMAPve_d_BCM_Right_Light_1 : DataTypeConversion  OutDataTypeStr=uint16
  IMAPve_d_BCM_Right_Light_2 : Terminator
  IMAPve_d_BCM_Trunk_State_1 : DataTypeConversion  OutDataTypeStr=uint16
  IMAPve_d_BCM_Trunk_State_2 : Terminator
  IMAPve_d_Brake_Pedal_Fault_1 : DataTypeConversion  OutDataTypeStr=uint16
  IMAPve_d_Brake_Pedal_Fault_2 : Terminator
  IMAPve_d_Camera_Signal_Fault_1 : DataTypeConversion  OutDataTypeStr=uint16
  IMAPve_d_Camera_Signal_Fault_2 : Terminator
  IMAPve_d_Camera_Status_1 : DataTypeConversion  OutDataTypeStr=uint16
  IMAPve_d_Camera_Status_2 : Terminator
  IMAPve_d_ConsArea_1 : DataTypeConversion  OutDataTypeStr=uint16
  IMAPve_d_ConsArea_2 : Terminator
  IMAPve_d_EMS_ACC_CtlAvail_1 : DataTypeConversion  OutDataTypeStr=uint16
  IMAPve_d_EMS_ACC_CtlAvail_2 : Terminator
  IMAPve_d_EMS_ACC_Effective_1 : DataTypeConversion  OutDataTypeStr=uint16
  IMAPve_d_EMS_ACC_Effective_2 : Terminator
  IMAPve_d_EMS_ACC_Inhibited_1 : DataTypeConversion  OutDataTypeStr=uint16
  IMAPve_d_EMS_ACC_Inhibited_2 : Terminator
  IMAPve_d_EMS_ACC_Status_1 : DataTypeConversion  OutDataTypeStr=uint16
  IMAPve_d_EMS_ACC_Status_2 : Terminator
  IMAPve_d_EMS_AccPedal_Fault_1 : DataTypeConversion  OutDataTypeStr=uint16
  IMAPve_d_EMS_AccPedal_Fault_2 : Terminator
  IMAPve_d_EMS_Brake_Pedal_1 : DataTypeConversion  OutDataTypeStr=uint16
  IMAPve_d_EMS_Brake_Pedal_2 : Terminator
  IMAPve_d_EMS_Engine_Status_1 : DataTypeConversion  OutDataTypeStr=uint16
  IMAPve_d_EMS_Engine_Status_2 : Terminator
  IMAPve_d_EMS_Gearbox_CtlAvail_1 : DataTypeConversion  OutDataTypeStr=uint16
  IMAPve_d_EMS_Gearbox_CtlAvail_2 : Terminator
  IMAPve_d_EPB_Display_Req_1 : DataTypeConversion  OutDataTypeStr=uint16
  IMAPve_d_EPB_Display_Req_2 : Terminator
  IMAPve_d_EPB_Status_1 : DataTypeConversion  OutDataTypeStr=uint16
  IMAPve_d_EPB_Status_2 : Terminator
  IMAPve_d_EPB_Switch_State_1 : DataTypeConversion  OutDataTypeStr=uint16
  IMAPve_d_EPB_Switch_State_2 : Terminator
  IMAPve_d_EPB_Switch_Valid_1 : DataTypeConversion  OutDataTypeStr=uint16
  IMAPve_d_EPB_Switch_Valid_2 : Terminator
  IMAPve_d_EPB_Warn_Req_1 : DataTypeConversion  OutDataTypeStr=uint16
  IMAPve_d_EPB_Warn_Req_2 : Terminator
  IMAPve_d_EPS_Error_State_1 : DataTypeConversion  OutDataTypeStr=uint16
  IMAPve_d_EPS_Error_State_2 : Terminator
  IMAPve_d_EPS_LKA_State_1 : DataTypeConversion  OutDataTypeStr=uint16
  IMAPve_d_EPS_LKA_State_2 : Terminator
  IMAPve_d_EPS_Steer_Hold_State_1 : DataTypeConversion  OutDataTypeStr=uint16
  IMAPve_d_EPS_Steer_Hold_State_2 : Terminator
  IMAPve_d_EPS_TrqLim_State_1 : DataTypeConversion  OutDataTypeStr=uint16
  IMAPve_d_EPS_TrqLim_State_2 : Terminator
  IMAPve_d_EPS_Trq_State_1 : DataTypeConversion  OutDataTypeStr=uint16
  IMAPve_d_EPS_Trq_State_2 : Terminator
  IMAPve_d_EPS_Warning_State_1 : DataTypeConversion  OutDataTypeStr=uint16
  IMAPve_d_EPS_Warning_State_2 : Terminator
  IMAPve_d_ESC_ABS_Active_1 : DataTypeConversion  OutDataTypeStr=uint16
  IMAPve_d_ESC_ABS_Active_2 : Terminator
  IMAPve_d_ESC_ABS_AlarmSig_1 : DataTypeConversion  OutDataTypeStr=uint16
  IMAPve_d_ESC_ABS_AlarmSig_2 : Terminator
  IMAPve_d_ESC_ABS_Valid_1 : DataTypeConversion  OutDataTypeStr=uint16
  IMAPve_d_ESC_ABS_Valid_2 : Terminator
  IMAPve_d_ESC_ACC_Active_1 : DataTypeConversion  OutDataTypeStr=uint16
  IMAPve_d_ESC_ACC_Active_2 : Terminator
  IMAPve_d_ESC_ACC_Available_1 : DataTypeConversion  OutDataTypeStr=uint16
  IMAPve_d_ESC_ACC_Available_2 : Terminator
  IMAPve_d_ESC_ACC_Status_1 : DataTypeConversion  OutDataTypeStr=uint16
  IMAPve_d_ESC_ACC_Status_2 : Terminator
  IMAPve_d_ESC_AEB_Active_1 : DataTypeConversion  OutDataTypeStr=uint16
  IMAPve_d_ESC_AEB_Active_2 : Terminator
  IMAPve_d_ESC_AEB_Available_1 : DataTypeConversion  OutDataTypeStr=uint16
  IMAPve_d_ESC_AEB_Available_2 : Terminator
  IMAPve_d_ESC_AEB_Status_1 : DataTypeConversion  OutDataTypeStr=uint16
  IMAPve_d_ESC_AEB_Status_2 : Terminator
  IMAPve_d_ESC_AVH_Status_1 : DataTypeConversion  OutDataTypeStr=uint16
  IMAPve_d_ESC_AVH_Status_2 : Terminator
  IMAPve_d_ESC_AlarmSig_1 : DataTypeConversion  OutDataTypeStr=uint16
  IMAPve_d_ESC_AlarmSig_2 : Terminator
  IMAPve_d_ESC_BrakeLamp_Req_1 : DataTypeConversion  OutDataTypeStr=uint16
  IMAPve_d_ESC_BrakeLamp_Req_2 : Terminator
  IMAPve_d_ESC_Brake_Effort_1 : DataTypeConversion  OutDataTypeStr=uint16
  IMAPve_d_ESC_Brake_Effort_2 : Terminator
  IMAPve_d_ESC_Brake_Failsafe_1 : DataTypeConversion  OutDataTypeStr=uint16
  IMAPve_d_ESC_Brake_Failsafe_2 : Terminator
  IMAPve_d_ESC_Drive_Direction_1 : DataTypeConversion  OutDataTypeStr=uint16
  IMAPve_d_ESC_Drive_Direction_2 : Terminator
  IMAPve_d_ESC_EBD_AlarmSig_1 : DataTypeConversion  OutDataTypeStr=uint16
  IMAPve_d_ESC_EBD_AlarmSig_2 : Terminator
  IMAPve_d_ESC_ESC_Active_1 : DataTypeConversion  OutDataTypeStr=uint16
  IMAPve_d_ESC_ESC_Active_2 : Terminator
  IMAPve_d_ESC_FL_WheelPulVal_1 : DataTypeConversion  OutDataTypeStr=uint16
  IMAPve_d_ESC_FL_WheelPulVal_2 : Terminator
  IMAPve_d_ESC_FL_Wheel_Pulse_1 : DataTypeConversion  OutDataTypeStr=uint16
  IMAPve_d_ESC_FL_Wheel_Pulse_2 : Terminator
  IMAPve_d_ESC_FL_WhlSpd_Fault_1 : DataTypeConversion  OutDataTypeStr=uint16
  IMAPve_d_ESC_FL_WhlSpd_Fault_2 : Terminator
  IMAPve_d_ESC_FR_WheelPulVal_1 : DataTypeConversion  OutDataTypeStr=uint16
  IMAPve_d_ESC_FR_WheelPulVal_2 : Terminator
  IMAPve_d_ESC_FR_Wheel_Pulse_1 : DataTypeConversion  OutDataTypeStr=uint16
  IMAPve_d_ESC_FR_Wheel_Pulse_2 : Terminator
  IMAPve_d_ESC_FR_WhlSpd_Fault_1 : DataTypeConversion  OutDataTypeStr=uint16
  IMAPve_d_ESC_FR_WhlSpd_Fault_2 : Terminator
  IMAPve_d_ESC_Hold_State_1 : DataTypeConversion  OutDataTypeStr=uint16
  IMAPve_d_ESC_Hold_State_2 : Terminator
  IMAPve_d_ESC_LatAcc_Valid_1 : DataTypeConversion  OutDataTypeStr=uint16
  IMAPve_d_ESC_LatAcc_Valid_2 : Terminator
  IMAPve_d_ESC_LonAcc_Valid_1 : DataTypeConversion  OutDataTypeStr=uint16
  IMAPve_d_ESC_LonAcc_Valid_2 : Terminator
  IMAPve_d_ESC_MSR_Active_1 : DataTypeConversion  OutDataTypeStr=uint16
  IMAPve_d_ESC_MSR_Active_2 : Terminator
  IMAPve_d_ESC_OFF_1 : DataTypeConversion  OutDataTypeStr=uint16
  IMAPve_d_ESC_OFF_2 : Terminator
  IMAPve_d_ESC_RL_WheelPulVal_1 : DataTypeConversion  OutDataTypeStr=uint16
  IMAPve_d_ESC_RL_WheelPulVal_2 : Terminator
  IMAPve_d_ESC_RL_Wheel_Pulse_1 : DataTypeConversion  OutDataTypeStr=uint16
  IMAPve_d_ESC_RL_Wheel_Pulse_2 : Terminator
  IMAPve_d_ESC_RL_WhlSpd_Fault_1 : DataTypeConversion  OutDataTypeStr=uint16
  IMAPve_d_ESC_RL_WhlSpd_Fault_2 : Terminator
  IMAPve_d_ESC_RR_WheelPulVal_1 : DataTypeConversion  OutDataTypeStr=uint16
  IMAPve_d_ESC_RR_WheelPulVal_2 : Terminator
  IMAPve_d_ESC_RR_Wheel_Pulse_1 : DataTypeConversion  OutDataTypeStr=uint16
  IMAPve_d_ESC_RR_Wheel_Pulse_2 : Terminator
  IMAPve_d_ESC_RR_WhlSpd_Fault_1 : DataTypeConversion  OutDataTypeStr=uint16
  IMAPve_d_ESC_RR_WhlSpd_Fault_2 : Terminator
  IMAPve_d_ESC_TCS_Active_1 : DataTypeConversion  OutDataTypeStr=uint16
  IMAPve_d_ESC_TCS_Active_2 : Terminator
  IMAPve_d_ESC_VehSpd_Valid_1 : DataTypeConversion  OutDataTypeStr=uint16
  IMAPve_d_ESC_VehSpd_Valid_2 : Terminator
  IMAPve_d_ESC_Veh_Standstill_1 : DataTypeConversion  OutDataTypeStr=uint16
  IMAPve_d_ESC_Veh_Standstill_2 : Terminator
  IMAPve_d_ESC_YawRate_Valid_1 : DataTypeConversion  OutDataTypeStr=uint16
  IMAPve_d_ESC_YawRate_Valid_2 : Terminator
  IMAPve_d_Fusion_Status_1 : DataTypeConversion  OutDataTypeStr=uint16
  IMAPve_d_Fusion_Status_2 : Terminator
  IMAPve_d_GW_Brake_Only_Req_1 : DataTypeConversion  OutDataTypeStr=uint16
  IMAPve_d_GW_Brake_Only_Req_2 : Terminator
  IMAPve_d_L0_LC_1 : DataTypeConversion  OutDataTypeStr=uint16
  IMAPve_d_L0_LC_2 : Terminator
  IMAPve_d_L0_Q_1 : DataTypeConversion  OutDataTypeStr=uint16
  IMAPve_d_L0_Q_2 : Terminator
  IMAPve_d_L0_Type_1 : DataTypeConversion  OutDataTypeStr=uint16
  IMAPve_d_L0_Type_2 : Terminator
  IMAPve_d_L1_LC_1 : DataTypeConversion  OutDataTypeStr=uint16
  IMAPve_d_L1_LC_2 : Terminator
  IMAPve_d_L1_Q_1 : DataTypeConversion  OutDataTypeStr=uint16
  IMAPve_d_L1_Q_2 : Terminator
  IMAPve_d_L1_Type_1 : DataTypeConversion  OutDataTypeStr=uint16
  IMAPve_d_L1_Type_2 : Terminator
  IMAPve_d_LF_Radar_Status_1 : DataTypeConversion  OutDataTypeStr=uint16
  IMAPve_d_LF_Radar_Status_2 : Terminator
  IMAPve_d_LR_Radar_Status_1 : DataTypeConversion  OutDataTypeStr=uint16
  IMAPve_d_LR_Radar_Status_2 : Terminator
  IMAPve_d_Lane_Valid_1 : DataTypeConversion  OutDataTypeStr=uint16
  IMAPve_d_Lane_Valid_2 : Terminator
  IMAPve_d_ORI_CIPV_ID_1 : DataTypeConversion  OutDataTypeStr=uint16
  IMAPve_d_ORI_CIPV_ID_2 : Terminator
  IMAPve_d_ORI_L0_LC_1 : DataTypeConversion  OutDataTypeStr=uint16
  IMAPve_d_ORI_L0_LC_2 : Terminator
  IMAPve_d_ORI_L0_Q_1 : DataTypeConversion  OutDataTypeStr=uint16
  IMAPve_d_ORI_L0_Q_2 : Terminator
  IMAPve_d_ORI_L0_Type_1 : DataTypeConversion  OutDataTypeStr=uint16
  IMAPve_d_ORI_L0_Type_2 : Terminator
  IMAPve_d_ORI_L1_LC_1 : DataTypeConversion  OutDataTypeStr=uint16
  IMAPve_d_ORI_L1_LC_2 : Terminator
  IMAPve_d_ORI_L1_Q_1 : DataTypeConversion  OutDataTypeStr=uint16
  IMAPve_d_ORI_L1_Q_2 : Terminator
  IMAPve_d_ORI_L1_Type_1 : DataTypeConversion  OutDataTypeStr=uint16
  IMAPve_d_ORI_L1_Type_2 : Terminator
  IMAPve_d_ORI_Lane_ConsArea_1 : DataTypeConversion  OutDataTypeStr=uint16
  IMAPve_d_ORI_Lane_ConsArea_2 : Terminator
  IMAPve_d_ORI_Lane_RoadType_1 : DataTypeConversion  OutDataTypeStr=uint16
  IMAPve_d_ORI_Lane_RoadType_2 : Terminator
  IMAPve_d_ORI_Lane_Valid_1 : DataTypeConversion  OutDataTypeStr=uint16
  IMAPve_d_ORI_Lane_Valid_2 : Terminator
  IMAPve_d_ORI_Obj_Num_1 : DataTypeConversion  OutDataTypeStr=uint16
  IMAPve_d_ORI_Obj_Num_2 : Terminator
  IMAPve_d_ORI_R0_LC_1 : DataTypeConversion  OutDataTypeStr=uint16
  IMAPve_d_ORI_R0_LC_2 : Terminator
  IMAPve_d_ORI_R0_LT_1 : DataTypeConversion  OutDataTypeStr=uint16
  IMAPve_d_ORI_R0_LT_2 : Terminator
  IMAPve_d_ORI_R0_Q_1 : DataTypeConversion  OutDataTypeStr=uint16
  IMAPve_d_ORI_R0_Q_2 : Terminator
  IMAPve_d_ORI_R1_LC_1 : DataTypeConversion  OutDataTypeStr=uint16
  IMAPve_d_ORI_R1_LC_2 : Terminator
  IMAPve_d_ORI_R1_LT_1 : DataTypeConversion  OutDataTypeStr=uint16
  IMAPve_d_ORI_R1_LT_2 : Terminator
  IMAPve_d_ORI_R1_Q_1 : DataTypeConversion  OutDataTypeStr=uint16
  IMAPve_d_ORI_R1_Q_2 : Terminator
  IMAPve_d_Outside_Temp_1 : DataTypeConversion  OutDataTypeStr=uint16
  IMAPve_d_Outside_Temp_2 : Terminator
  IMAPve_d_PEPS_Door_Lock_Req_1 : DataTypeConversion  OutDataTypeStr=uint16
  IMAPve_d_PEPS_Door_Lock_Req_2 : Terminator
  IMAPve_d_R0_LC_1 : DataTypeConversion  OutDataTypeStr=uint16
  IMAPve_d_R0_LC_2 : Terminator
  IMAPve_d_R0_Q_1 : DataTypeConversion  OutDataTypeStr=uint16
  IMAPve_d_R0_Q_2 : Terminator
  IMAPve_d_R0_Type_1 : DataTypeConversion  OutDataTypeStr=uint16
  IMAPve_d_R0_Type_2 : Terminator
  IMAPve_d_R1_LC_1 : DataTypeConversion  OutDataTypeStr=uint16
  IMAPve_d_R1_LC_2 : Terminator
  IMAPve_d_R1_Q_1 : DataTypeConversion  OutDataTypeStr=uint16
  IMAPve_d_R1_Q_2 : Terminator
  IMAPve_d_R1_Type_1 : DataTypeConversion  OutDataTypeStr=uint16
  IMAPve_d_R1_Type_2 : Terminator
  IMAPve_d_RF_Radar_Status_1 : DataTypeConversion  OutDataTypeStr=uint16
  IMAPve_d_RF_Radar_Status_2 : Terminator
  IMAPve_d_RR_Radar_Status_1 : DataTypeConversion  OutDataTypeStr=uint16
  IMAPve_d_RR_Radar_Status_2 : Terminator
  IMAPve_d_Radar_Detective_Req_1 : DataTypeConversion  OutDataTypeStr=uint16
  IMAPve_d_Radar_Detective_Req_2 : Terminator
  IMAPve_d_Radar_State_1 : DataTypeConversion  OutDataTypeStr=uint16
  IMAPve_d_Radar_State_2 : Terminator
  IMAPve_d_Radar_Status_1 : DataTypeConversion  OutDataTypeStr=uint16
  IMAPve_d_Radar_Status_2 : Terminator
  IMAPve_d_Road_Type_1 : DataTypeConversion  OutDataTypeStr=uint16
  IMAPve_d_Road_Type_2 : Terminator
  IMAPve_d_SAS_Clb_State_1 : DataTypeConversion  OutDataTypeStr=uint16
  IMAPve_d_SAS_Clb_State_2 : Terminator
  IMAPve_d_SAS_Trim_State_1 : DataTypeConversion  OutDataTypeStr=uint16
  IMAPve_d_SAS_Trim_State_2 : Terminator
  IMAPve_d_SCC_Left_SwitchSig_1 : DataTypeConversion  OutDataTypeStr=uint16
  IMAPve_d_SCC_Left_SwitchSig_2 : Terminator
  IMAPve_d_SCC_Right_SwitchSig_1 : DataTypeConversion  OutDataTypeStr=uint16
  IMAPve_d_SCC_Right_SwitchSig_2 : Terminator
  IMAPve_d_SWS_Failure_Status_1 : DataTypeConversion  OutDataTypeStr=uint16
  IMAPve_d_SWS_Failure_Status_2 : Terminator
  IMAPve_d_SWS_Fault_Code_1 : DataTypeConversion  OutDataTypeStr=uint16
  IMAPve_d_SWS_Fault_Code_2 : Terminator
  IMAPve_d_Sensor_Status_1 : DataTypeConversion  OutDataTypeStr=uint16
  IMAPve_d_Sensor_Status_2 : Terminator
  IMAPve_d_Sign_ISA_Value_1 : DataTypeConversion  OutDataTypeStr=uint16
  IMAPve_d_Sign_ISA_Value_2 : Terminator
  IMAPve_d_Signal_Time_Stamp_1 : DataTypeConversion  OutDataTypeStr=uint16
  IMAPve_d_Signal_Time_Stamp_2 : Terminator
  IMAPve_d_Speed_Limit_Switch_1 : DataTypeConversion  OutDataTypeStr=uint16
  IMAPve_d_Speed_Limit_Switch_2 : Terminator
  IMAPve_d_TBOX_LocalTimeD_1 : DataTypeConversion  OutDataTypeStr=uint16
  IMAPve_d_TBOX_LocalTimeD_2 : Terminator
  IMAPve_d_TBOX_LocalTimeH_1 : DataTypeConversion  OutDataTypeStr=uint16
  IMAPve_d_TBOX_LocalTimeH_2 : Terminator
  IMAPve_d_TBOX_LocalTimeM_1 : DataTypeConversion  OutDataTypeStr=uint16
  IMAPve_d_TBOX_LocalTimeM_2 : Terminator
  IMAPve_d_TBOX_LocalTimeMin_1 : DataTypeConversion  OutDataTypeStr=uint16
  IMAPve_d_TBOX_LocalTimeMin_2 : Terminator
  IMAPve_d_TBOX_LocalTimeS_1 : DataTypeConversion  OutDataTypeStr=uint16
  IMAPve_d_TBOX_LocalTimeS_2 : Terminator
  IMAPve_d_TBOX_LocalTimeY_1 : DataTypeConversion  OutDataTypeStr=uint16
  IMAPve_d_TBOX_LocalTimeY_2 : Terminator
  IMAPve_d_TBOX_LocalTime_Valid_1 : DataTypeConversion  OutDataTypeStr=uint16
  IMAPve_d_TBOX_LocalTime_Valid_2 : Terminator
  IMAPve_d_TCU_AT_Failure_1 : DataTypeConversion  OutDataTypeStr=uint16
  IMAPve_d_TCU_AT_Failure_2 : Terminator
  IMAPve_d_TCU_Actual_Gear_1 : DataTypeConversion  OutDataTypeStr=uint16
  IMAPve_d_TCU_Actual_Gear_2 : Terminator
  IMAPve_d_TCU_DCT_Clutch_State_1 : DataTypeConversion  OutDataTypeStr=uint16
  IMAPve_d_TCU_DCT_Clutch_State_2 : Terminator
  IMAPve_d_TCU_Gear_Engage_1 : DataTypeConversion  OutDataTypeStr=uint16
  IMAPve_d_TCU_Gear_Engage_2 : Terminator
  IMAPve_d_TCU_PRND_State_1 : DataTypeConversion  OutDataTypeStr=uint16
  IMAPve_d_TCU_PRND_State_2 : Terminator
  IMAPve_d_TCU_Select_ATMode_1 : DataTypeConversion  OutDataTypeStr=uint16
  IMAPve_d_TCU_Select_ATMode_2 : Terminator
  IMAPve_d_TCU_Shift_Valid_1 : DataTypeConversion  OutDataTypeStr=uint16
  IMAPve_d_TCU_Shift_Valid_2 : Terminator
  IMAPve_d_TCU_Target_Gear_1 : DataTypeConversion  OutDataTypeStr=uint16
  IMAPve_d_TCU_Target_Gear_2 : Terminator
  IMAPve_d_TPMS_Warn_Indicate_1 : DataTypeConversion  OutDataTypeStr=uint16
  IMAPve_d_TPMS_Warn_Indicate_2 : Terminator
  IMAPve_d_TSR_Sign_Type_1 : DataTypeConversion  OutDataTypeStr=uint16
  IMAPve_d_TSR_Sign_Type_2 : Terminator
  IMAPve_d_Time_System_Clock_1 : DataTypeConversion  OutDataTypeStr=uint16
  IMAPve_d_Time_System_Clock_2 : Terminator
  IMAPve_d_obj_Num_1 : DataTypeConversion  OutDataTypeStr=uint16
  IMAPve_d_obj_Num_2 : Terminator
  IMAPve_g_BCM_Battery_Voltage_1 : DataTypeConversion  OutDataTypeStr=single
  IMAPve_g_BCM_Battery_Voltage_2 : Terminator
  IMAPve_g_EMS_ACC_VirtualPedal_1 : DataTypeConversion  OutDataTypeStr=single
  IMAPve_g_EMS_ACC_VirtualPedal_2 : Terminator
  IMAPve_g_EMS_Actual_FlwT_1 : DataTypeConversion  OutDataTypeStr=single
  IMAPve_g_EMS_Actual_FlwT_2 : Terminator
  IMAPve_g_EMS_Actual_IndT_1 : DataTypeConversion  OutDataTypeStr=single
  IMAPve_g_EMS_Actual_IndT_2 : Terminator
  IMAPve_g_EMS_Driver_Torque_1 : DataTypeConversion  OutDataTypeStr=single
  IMAPve_g_EMS_Driver_Torque_2 : Terminator
  IMAPve_g_EMS_Engine_Speed_1 : DataTypeConversion  OutDataTypeStr=single
  IMAPve_g_EMS_Engine_Speed_2 : Terminator
  IMAPve_g_EMS_MaxTWhl_1 : DataTypeConversion  OutDataTypeStr=single
  IMAPve_g_EMS_MaxTWhl_2 : Terminator
  IMAPve_g_EMS_MaxTWhl_Offset_1 : DataTypeConversion  OutDataTypeStr=single
  IMAPve_g_EMS_MaxTWhl_Offset_2 : Terminator
  IMAPve_g_EMS_MinTWhl_1 : DataTypeConversion  OutDataTypeStr=single
  IMAPve_g_EMS_MinTWhl_2 : Terminator
  IMAPve_g_EMS_MinTWhl_Offset_1 : DataTypeConversion  OutDataTypeStr=single
  IMAPve_g_EMS_MinTWhl_Offset_2 : Terminator
  IMAPve_g_EMS_Pot_WhlT_Max_1 : DataTypeConversion  OutDataTypeStr=single
  IMAPve_g_EMS_Pot_WhlT_Max_2 : Terminator
  IMAPve_g_EMS_Pot_WhlT_Min_1 : DataTypeConversion  OutDataTypeStr=single
  IMAPve_g_EMS_Pot_WhlT_Min_2 : Terminator
  IMAPve_g_EMS_RealPedal_1 : DataTypeConversion  OutDataTypeStr=single
  IMAPve_g_EMS_RealPedal_2 : Terminator
  IMAPve_g_EMS_Realize_TWhl_1 : DataTypeConversion  OutDataTypeStr=single
  IMAPve_g_EMS_Realize_TWhl_2 : Terminator
  IMAPve_g_EPS_LKA_Current_1 : DataTypeConversion  OutDataTypeStr=single
  IMAPve_g_EPS_LKA_Current_2 : Terminator
  IMAPve_g_EPS_PowerCon_1 : DataTypeConversion  OutDataTypeStr=single
  IMAPve_g_EPS_PowerCon_2 : Terminator
  IMAPve_g_EPS_SW_Trq_1 : DataTypeConversion  OutDataTypeStr=single
  IMAPve_g_EPS_SW_Trq_2 : Terminator
  IMAPve_g_ESC_Brake_Press_1 : DataTypeConversion  OutDataTypeStr=single
  IMAPve_g_ESC_Brake_Press_2 : Terminator
  IMAPve_g_ESC_DySlope_1 : DataTypeConversion  OutDataTypeStr=single
  IMAPve_g_ESC_DySlope_2 : Terminator
  IMAPve_g_ESC_DySlope_Accuracy_1 : DataTypeConversion  OutDataTypeStr=single
  IMAPve_g_ESC_DySlope_Accuracy_2 : Terminator
  IMAPve_g_ESC_FL_WhlSpd_1 : DataTypeConversion  OutDataTypeStr=single
  IMAPve_g_ESC_FL_WhlSpd_2 : Terminator
  IMAPve_g_ESC_FR_WhlSpd_1 : DataTypeConversion  OutDataTypeStr=single
  IMAPve_g_ESC_FR_WhlSpd_2 : Terminator
  IMAPve_g_ESC_LatAcc_1 : DataTypeConversion  OutDataTypeStr=single
  IMAPve_g_ESC_LatAcc_2 : Terminator
  IMAPve_g_ESC_LonAcc_1 : DataTypeConversion  OutDataTypeStr=single
  IMAPve_g_ESC_LonAcc_2 : Terminator
  IMAPve_g_ESC_RL_WhlSpd_1 : DataTypeConversion  OutDataTypeStr=single
  IMAPve_g_ESC_RL_WhlSpd_2 : Terminator
  IMAPve_g_ESC_RR_WhlSpd_1 : DataTypeConversion  OutDataTypeStr=single
  IMAPve_g_ESC_RR_WhlSpd_2 : Terminator
  IMAPve_g_ESC_Static_Slope_1 : DataTypeConversion  OutDataTypeStr=single
  IMAPve_g_ESC_Static_Slope_2 : Terminator
  IMAPve_g_ESC_UnYawRate_1 : DataTypeConversion  OutDataTypeStr=single
  IMAPve_g_ESC_UnYawRate_2 : Terminator
  IMAPve_g_ESC_VehSpd_1 : DataTypeConversion  OutDataTypeStr=single
  IMAPve_g_ESC_VehSpd_2 : Terminator
  IMAPve_g_ESC_YawRate_1 : DataTypeConversion  OutDataTypeStr=single
  IMAPve_g_ESC_YawRate_2 : Terminator
  IMAPve_g_FAPA_State_1 : DataTypeConversion  OutDataTypeStr=single
  IMAPve_g_FAPA_State_2 : Terminator
  IMAPve_g_Fusion_Time_Stamp_1 : DataTypeConversion  OutDataTypeStr=single
  IMAPve_g_Fusion_Time_Stamp_2 : Terminator
  IMAPve_g_GW_IC_Odometer_1 : DataTypeConversion  OutDataTypeStr=single
  IMAPve_g_GW_IC_Odometer_2 : Terminator
  IMAPve_g_L0_C0_1 : DataTypeConversion  OutDataTypeStr=single
  IMAPve_g_L0_C0_2 : Terminator
  IMAPve_g_L0_C0_Back_1 : DataTypeConversion  OutDataTypeStr=single
  IMAPve_g_L0_C0_Back_2 : Terminator
  IMAPve_g_L0_C0_FR_Pred_1 : DataTypeConversion  OutDataTypeStr=single
  IMAPve_g_L0_C0_FR_Pred_2 : Terminator
  IMAPve_g_L0_C1_1 : DataTypeConversion  OutDataTypeStr=single
  IMAPve_g_L0_C1_2 : Terminator
  IMAPve_g_L0_C1_Back_1 : DataTypeConversion  OutDataTypeStr=single
  IMAPve_g_L0_C1_Back_2 : Terminator
  IMAPve_g_L0_C1_FR_Pred_1 : DataTypeConversion  OutDataTypeStr=single
  IMAPve_g_L0_C1_FR_Pred_2 : Terminator
  IMAPve_g_L0_C2_1 : DataTypeConversion  OutDataTypeStr=single
  IMAPve_g_L0_C2_2 : Terminator
  IMAPve_g_L0_C2_Back_1 : DataTypeConversion  OutDataTypeStr=single
  IMAPve_g_L0_C2_Back_2 : Terminator
  IMAPve_g_L0_C2_FR_Pred_1 : DataTypeConversion  OutDataTypeStr=single
  IMAPve_g_L0_C2_FR_Pred_2 : Terminator
  IMAPve_g_L0_C3_1 : DataTypeConversion  OutDataTypeStr=single
  IMAPve_g_L0_C3_2 : Terminator
  IMAPve_g_L0_C3_Back_1 : DataTypeConversion  OutDataTypeStr=single
  IMAPve_g_L0_C3_Back_2 : Terminator
  IMAPve_g_L0_Confidence_1 : DataTypeConversion  OutDataTypeStr=single
  IMAPve_g_L0_Confidence_2 : Terminator
  IMAPve_g_L0_Range_Back_1 : DataTypeConversion  OutDataTypeStr=single
  IMAPve_g_L0_Range_Back_2 : Terminator
  IMAPve_g_L0_Range_FR_Pred_1 : DataTypeConversion  OutDataTypeStr=single
  IMAPve_g_L0_Range_FR_Pred_2 : Terminator
  IMAPve_g_L0_TLC_1 : DataTypeConversion  OutDataTypeStr=single
  IMAPve_g_L0_TLC_2 : Terminator
  IMAPve_g_L0_VR_1 : DataTypeConversion  OutDataTypeStr=single
  IMAPve_g_L0_VR_2 : Terminator
  IMAPve_g_L0_W_1 : DataTypeConversion  OutDataTypeStr=single
  IMAPve_g_L0_W_2 : Terminator
  IMAPve_g_L1_C0_1 : DataTypeConversion  OutDataTypeStr=single
  IMAPve_g_L1_C0_2 : Terminator
  IMAPve_g_L1_C0_Back_1 : DataTypeConversion  OutDataTypeStr=single
  IMAPve_g_L1_C0_Back_2 : Terminator
  IMAPve_g_L1_C0_FR_Pred_1 : DataTypeConversion  OutDataTypeStr=single
  IMAPve_g_L1_C0_FR_Pred_2 : Terminator
  IMAPve_g_L1_C1_1 : DataTypeConversion  OutDataTypeStr=single
  IMAPve_g_L1_C1_2 : Terminator
  IMAPve_g_L1_C1_Back_1 : DataTypeConversion  OutDataTypeStr=single
  IMAPve_g_L1_C1_Back_2 : Terminator
  IMAPve_g_L1_C1_FR_Pred_1 : DataTypeConversion  OutDataTypeStr=single
  IMAPve_g_L1_C1_FR_Pred_2 : Terminator
  IMAPve_g_L1_C2_1 : DataTypeConversion  OutDataTypeStr=single
  IMAPve_g_L1_C2_2 : Terminator
  IMAPve_g_L1_C2_Back_1 : DataTypeConversion  OutDataTypeStr=single
  IMAPve_g_L1_C2_Back_2 : Terminator
  IMAPve_g_L1_C2_FR_Pred_1 : DataTypeConversion  OutDataTypeStr=single
  IMAPve_g_L1_C2_FR_Pred_2 : Terminator
  IMAPve_g_L1_C3_1 : DataTypeConversion  OutDataTypeStr=single
  IMAPve_g_L1_C3_2 : Terminator
  IMAPve_g_L1_C3_Back_1 : DataTypeConversion  OutDataTypeStr=single
  IMAPve_g_L1_C3_Back_2 : Terminator
  IMAPve_g_L1_Confidence_1 : DataTypeConversion  OutDataTypeStr=single
  IMAPve_g_L1_Confidence_2 : Terminator
  IMAPve_g_L1_Range_Back_1 : DataTypeConversion  OutDataTypeStr=single
  IMAPve_g_L1_Range_Back_2 : Terminator
  IMAPve_g_L1_Range_FR_Pred_1 : DataTypeConversion  OutDataTypeStr=single
  IMAPve_g_L1_Range_FR_Pred_2 : Terminator
  IMAPve_g_L1_TLC_1 : DataTypeConversion  OutDataTypeStr=single
  IMAPve_g_L1_TLC_2 : Terminator
  IMAPve_g_L1_VR_1 : DataTypeConversion  OutDataTypeStr=single
  IMAPve_g_L1_VR_2 : Terminator
  IMAPve_g_L1_W_1 : DataTypeConversion  OutDataTypeStr=single
  IMAPve_g_L1_W_2 : Terminator
  IMAPve_g_ORI_L0_C0_1 : DataTypeConversion  OutDataTypeStr=single
  IMAPve_g_ORI_L0_C0_2 : Terminator
  IMAPve_g_ORI_L0_C1_1 : DataTypeConversion  OutDataTypeStr=single
  IMAPve_g_ORI_L0_C1_2 : Terminator
  IMAPve_g_ORI_L0_C2_1 : DataTypeConversion  OutDataTypeStr=single
  IMAPve_g_ORI_L0_C2_2 : Terminator
  IMAPve_g_ORI_L0_C3_1 : DataTypeConversion  OutDataTypeStr=single
  IMAPve_g_ORI_L0_C3_2 : Terminator
  IMAPve_g_ORI_L0_TLC_1 : DataTypeConversion  OutDataTypeStr=single
  IMAPve_g_ORI_L0_TLC_2 : Terminator
  IMAPve_g_ORI_L0_VR_1 : DataTypeConversion  OutDataTypeStr=single
  IMAPve_g_ORI_L0_VR_2 : Terminator
  IMAPve_g_ORI_L0_W_1 : DataTypeConversion  OutDataTypeStr=single
  IMAPve_g_ORI_L0_W_2 : Terminator
  IMAPve_g_ORI_L1_C0_1 : DataTypeConversion  OutDataTypeStr=single
  IMAPve_g_ORI_L1_C0_2 : Terminator
  IMAPve_g_ORI_L1_C1_1 : DataTypeConversion  OutDataTypeStr=single
  IMAPve_g_ORI_L1_C1_2 : Terminator
  IMAPve_g_ORI_L1_C2_1 : DataTypeConversion  OutDataTypeStr=single
  IMAPve_g_ORI_L1_C2_2 : Terminator
  IMAPve_g_ORI_L1_C3_1 : DataTypeConversion  OutDataTypeStr=single
  IMAPve_g_ORI_L1_C3_2 : Terminator
  IMAPve_g_ORI_L1_TLC_1 : DataTypeConversion  OutDataTypeStr=single
  IMAPve_g_ORI_L1_TLC_2 : Terminator
  IMAPve_g_ORI_L1_VR_1 : DataTypeConversion  OutDataTypeStr=single
  IMAPve_g_ORI_L1_VR_2 : Terminator
  IMAPve_g_ORI_L1_W_1 : DataTypeConversion  OutDataTypeStr=single
  IMAPve_g_ORI_L1_W_2 : Terminator
  IMAPve_g_ORI_R0_C0_1 : DataTypeConversion  OutDataTypeStr=single
  IMAPve_g_ORI_R0_C0_2 : Terminator
  IMAPve_g_ORI_R0_C1_1 : DataTypeConversion  OutDataTypeStr=single
  IMAPve_g_ORI_R0_C1_2 : Terminator
  IMAPve_g_ORI_R0_C2_1 : DataTypeConversion  OutDataTypeStr=single
  IMAPve_g_ORI_R0_C2_2 : Terminator
  IMAPve_g_ORI_R0_C3_1 : DataTypeConversion  OutDataTypeStr=single
  IMAPve_g_ORI_R0_C3_2 : Terminator
  IMAPve_g_ORI_R0_TLC_1 : DataTypeConversion  OutDataTypeStr=single
  IMAPve_g_ORI_R0_TLC_2 : Terminator
  IMAPve_g_ORI_R0_VR_1 : DataTypeConversion  OutDataTypeStr=single
  IMAPve_g_ORI_R0_VR_2 : Terminator
  IMAPve_g_ORI_R0_W_1 : DataTypeConversion  OutDataTypeStr=single
  IMAPve_g_ORI_R0_W_2 : Terminator
  IMAPve_g_ORI_R1_C0_1 : DataTypeConversion  OutDataTypeStr=single
  IMAPve_g_ORI_R1_C0_2 : Terminator
  IMAPve_g_ORI_R1_C1_1 : DataTypeConversion  OutDataTypeStr=single
  IMAPve_g_ORI_R1_C1_2 : Terminator
  IMAPve_g_ORI_R1_C2_1 : DataTypeConversion  OutDataTypeStr=single
  IMAPve_g_ORI_R1_C2_2 : Terminator
  IMAPve_g_ORI_R1_C3_1 : DataTypeConversion  OutDataTypeStr=single
  IMAPve_g_ORI_R1_C3_2 : Terminator
  IMAPve_g_ORI_R1_TLC_1 : DataTypeConversion  OutDataTypeStr=single
  IMAPve_g_ORI_R1_TLC_2 : Terminator
  IMAPve_g_ORI_R1_VR_1 : DataTypeConversion  OutDataTypeStr=single
  IMAPve_g_ORI_R1_VR_2 : Terminator
  IMAPve_g_ORI_R1_W_1 : DataTypeConversion  OutDataTypeStr=single
  IMAPve_g_ORI_R1_W_2 : Terminator
  IMAPve_g_R0_C0_1 : DataTypeConversion  OutDataTypeStr=single
  IMAPve_g_R0_C0_2 : Terminator
  IMAPve_g_R0_C0_Back_1 : DataTypeConversion  OutDataTypeStr=single
  IMAPve_g_R0_C0_Back_2 : Terminator
  IMAPve_g_R0_C0_FR_Pred_1 : DataTypeConversion  OutDataTypeStr=single
  IMAPve_g_R0_C0_FR_Pred_2 : Terminator
  IMAPve_g_R0_C1_1 : DataTypeConversion  OutDataTypeStr=single
  IMAPve_g_R0_C1_2 : Terminator
  IMAPve_g_R0_C1_Back_1 : DataTypeConversion  OutDataTypeStr=single
  IMAPve_g_R0_C1_Back_2 : Terminator
  IMAPve_g_R0_C1_FR_Pred_1 : DataTypeConversion  OutDataTypeStr=single
  IMAPve_g_R0_C1_FR_Pred_2 : Terminator
  IMAPve_g_R0_C2_1 : DataTypeConversion  OutDataTypeStr=single
  IMAPve_g_R0_C2_2 : Terminator
  IMAPve_g_R0_C2_Back_1 : DataTypeConversion  OutDataTypeStr=single
  IMAPve_g_R0_C2_Back_2 : Terminator
  IMAPve_g_R0_C2_FR_Pred_1 : DataTypeConversion  OutDataTypeStr=single
  IMAPve_g_R0_C2_FR_Pred_2 : Terminator
  IMAPve_g_R0_C3_1 : DataTypeConversion  OutDataTypeStr=single
  IMAPve_g_R0_C3_2 : Terminator
  IMAPve_g_R0_C3_Back_1 : DataTypeConversion  OutDataTypeStr=single
  IMAPve_g_R0_C3_Back_2 : Terminator
  IMAPve_g_R0_Confidence_1 : DataTypeConversion  OutDataTypeStr=single
  IMAPve_g_R0_Confidence_2 : Terminator
  IMAPve_g_R0_Range_Back_1 : DataTypeConversion  OutDataTypeStr=single
  IMAPve_g_R0_Range_Back_2 : Terminator
  IMAPve_g_R0_Range_FR_Pred_1 : DataTypeConversion  OutDataTypeStr=single
  IMAPve_g_R0_Range_FR_Pred_2 : Terminator
  IMAPve_g_R0_TLC_1 : DataTypeConversion  OutDataTypeStr=single
  IMAPve_g_R0_TLC_2 : Terminator
  IMAPve_g_R0_VR_1 : DataTypeConversion  OutDataTypeStr=single
  IMAPve_g_R0_VR_2 : Terminator
  IMAPve_g_R0_W_1 : DataTypeConversion  OutDataTypeStr=single
  IMAPve_g_R0_W_2 : Terminator
  IMAPve_g_R1_C0_1 : DataTypeConversion  OutDataTypeStr=single
  IMAPve_g_R1_C0_2 : Terminator
  IMAPve_g_R1_C0_Back_1 : DataTypeConversion  OutDataTypeStr=single
  IMAPve_g_R1_C0_Back_2 : Terminator
  IMAPve_g_R1_C0_FR_Pred_1 : DataTypeConversion  OutDataTypeStr=single
  IMAPve_g_R1_C0_FR_Pred_2 : Terminator
  IMAPve_g_R1_C1_1 : DataTypeConversion  OutDataTypeStr=single
  IMAPve_g_R1_C1_2 : Terminator
  IMAPve_g_R1_C1_Back_1 : DataTypeConversion  OutDataTypeStr=single
  IMAPve_g_R1_C1_Back_2 : Terminator
  IMAPve_g_R1_C1_FR_Pred_1 : DataTypeConversion  OutDataTypeStr=single
  IMAPve_g_R1_C1_FR_Pred_2 : Terminator
  IMAPve_g_R1_C2_1 : DataTypeConversion  OutDataTypeStr=single
  IMAPve_g_R1_C2_2 : Terminator
  IMAPve_g_R1_C2_Back_1 : DataTypeConversion  OutDataTypeStr=single
  IMAPve_g_R1_C2_Back_2 : Terminator
  IMAPve_g_R1_C2_FR_Pred_1 : DataTypeConversion  OutDataTypeStr=single
  IMAPve_g_R1_C2_FR_Pred_2 : Terminator
  IMAPve_g_R1_C3_1 : DataTypeConversion  OutDataTypeStr=single
  IMAPve_g_R1_C3_2 : Terminator
  IMAPve_g_R1_C3_Back_1 : DataTypeConversion  OutDataTypeStr=single
  IMAPve_g_R1_C3_Back_2 : Terminator
  IMAPve_g_R1_Confidence_1 : DataTypeConversion  OutDataTypeStr=single
  IMAPve_g_R1_Confidence_2 : Terminator
  IMAPve_g_R1_Range_Back_1 : DataTypeConversion  OutDataTypeStr=single
  IMAPve_g_R1_Range_Back_2 : Terminator
  IMAPve_g_R1_Range_FR_Pred_1 : DataTypeConversion  OutDataTypeStr=single
  IMAPve_g_R1_Range_FR_Pred_2 : Terminator
  IMAPve_g_R1_TLC_1 : DataTypeConversion  OutDataTypeStr=single
  IMAPve_g_R1_TLC_2 : Terminator
  IMAPve_g_R1_VR_1 : DataTypeConversion  OutDataTypeStr=single
  IMAPve_g_R1_VR_2 : Terminator
  IMAPve_g_R1_W_1 : DataTypeConversion  OutDataTypeStr=single
  IMAPve_g_R1_W_2 : Terminator
  IMAPve_g_SW_Angle_1 : DataTypeConversion  OutDataTypeStr=single
  IMAPve_g_SW_Angle_2 : Terminator
  IMAPve_g_SW_Angle_Speed_1 : DataTypeConversion  OutDataTypeStr=single
  IMAPve_g_SW_Angle_Speed_2 : Terminator
  System_Clock1 : Terminator
  System_Clock_1 : DataTypeConversion  OutDataTypeStr=uint16
  ICACve_g_SteerAngleCmd : Outport
  ICACve_d_SteerAngleVld : Outport  Port=2
  ICACve_d_SignalTStamp : Outport  Port=3
  wires:
  System_Clock/1 -> System_Clock_1/1  "System_Clock"
  System_Clock_1/1 -> System_Clock1/1  "System_Clock"
  ICABva_g_VehParameter/1 -> ICABva_g_VehParameter_1/1  "ICABva_g_VehParameter"
  ICABva_g_VehParameter_1/1 -> ICABva_g_VehParameter1/1  "ICABva_g_VehParameter"
  ICABva_g_FilterInfo/1 -> ICABva_g_FilterInfo_1/1
  ICABva_g_FilterInfo_1/1 -> ICABva_g_FilterInfo_2/1
  ICABve_d_SignalTStamp/1 -> ICABve_d_SignalTStamp_1/1
  ICABve_d_SignalTStamp_1/1 -> ICABve_d_SignalTStamp_2/1
  ICAPva_g_PathPoints/1 -> ICAPva_g_PathPoints_1/1
  ICAPva_g_PathPoints_1/1 -> ICAPva_g_PathPoints_2/1
  ICAPve_d_PathPointNum/1 -> ICAPve_d_PathPointNum_1/1
  ICAPve_d_PathPointNum_1/1 -> ICAPve_d_PathPointNum_2/1
  ICAPve_d_PathValid/1 -> ICAPve_d_PathValid_1/1
  ICAPve_d_PathValid_1/1 -> ICAPve_d_PathValid_2/1
  ICAPve_d_SignalTStamp/1 -> ICAPve_d_SignalTStamp_1/1
  ICAPve_d_SignalTStamp_1/1 -> ICAPve_d_SignalTStamp_2/1
  ICASva_g_TrajectoryPoints/1 -> ICASva_g_TrajectoryPoints_1/1
  ICASva_g_TrajectoryPoints_1/1 -> ICASva_g_TrajectoryPoints_2/1
  ICASve_d_TrajectoryPointNum/1 -> ICASve_d_TrajectoryPointNum_1/1
  ICASve_d_TrajectoryPointNum_1/1 -> ICASve_d_TrajectoryPointNum_2/1
  ICASve_d_TrajectoryValid/1 -> ICASve_d_TrajectoryValid_1/1
  ICASve_d_TrajectoryValid_1/1 -> ICASve_d_TrajectoryValid_2/1
  ICASva_d_TrajectoryPlanState/1 -> ICASva_d_TrajectoryPlanState_1/1
  ICASva_d_TrajectoryPlanState_1/1 -> ICASva_d_TrajectoryPlanState_2/1
  ICASve_g_ExpLonAcc/1 -> ICASve_g_ExpLonAcc_1/1
  ICASve_g_ExpLonAcc_1/1 -> ICASve_g_ExpLonAcc_2/1
  ICASve_d_SignalTStamp/1 -> ICASve_d_SignalTStamp_1/1
  ICASve_d_SignalTStamp_1/1 -> ICASve_d_SignalTStamp_2/1
  IMAPve_d_EPS_LKA_State/1 -> IMAPve_d_EPS_LKA_State_1/1
  IMAPve_d_EPS_LKA_State_1/1 -> IMAPve_d_EPS_LKA_State_2/1
  IMAPve_g_EPS_SW_Trq/1 -> IMAPve_g_EPS_SW_Trq_1/1
  IMAPve_g_EPS_SW_Trq_1/1 -> IMAPve_g_EPS_SW_Trq_2/1
  IMAPve_d_EPS_Error_State/1 -> IMAPve_d_EPS_Error_State_1/1
  IMAPve_d_EPS_Error_State_1/1 -> IMAPve_d_EPS_Error_State_2/1
  IMAPve_d_EPS_Trq_State/1 -> IMAPve_d_EPS_Trq_State_1/1
  IMAPve_d_EPS_Trq_State_1/1 -> IMAPve_d_EPS_Trq_State_2/1
  IMAPve_d_SAS_Clb_State/1 -> IMAPve_d_SAS_Clb_State_1/1
  IMAPve_d_SAS_Clb_State_1/1 -> IMAPve_d_SAS_Clb_State_2/1
  IMAPve_d_SAS_Trim_State/1 -> IMAPve_d_SAS_Trim_State_1/1
  IMAPve_d_SAS_Trim_State_1/1 -> IMAPve_d_SAS_Trim_State_2/1
  IMAPve_d_EPS_TrqLim_State/1 -> IMAPve_d_EPS_TrqLim_State_1/1
  IMAPve_d_EPS_TrqLim_State_1/1 -> IMAPve_d_EPS_TrqLim_State_2/1
  IMAPve_g_EPS_LKA_Current/1 -> IMAPve_g_EPS_LKA_Current_1/1
  IMAPve_g_EPS_LKA_Current_1/1 -> IMAPve_g_EPS_LKA_Current_2/1
  IMAPve_g_ESC_LatAcc/1 -> IMAPve_g_ESC_LatAcc_1/1
  IMAPve_g_ESC_LatAcc_1/1 -> IMAPve_g_ESC_LatAcc_2/1
  IMAPve_d_ESC_LatAcc_Valid/1 -> IMAPve_d_ESC_LatAcc_Valid_1/1
  IMAPve_d_ESC_LatAcc_Valid_1/1 -> IMAPve_d_ESC_LatAcc_Valid_2/1
  IMAPve_g_ESC_YawRate/1 -> IMAPve_g_ESC_YawRate_1/1
  IMAPve_g_ESC_YawRate_1/1 -> IMAPve_g_ESC_YawRate_2/1
  IMAPve_d_ESC_YawRate_Valid/1 -> IMAPve_d_ESC_YawRate_Valid_1/1
  IMAPve_d_ESC_YawRate_Valid_1/1 -> IMAPve_d_ESC_YawRate_Valid_2/1
  IMAPve_g_ESC_UnYawRate/1 -> IMAPve_g_ESC_UnYawRate_1/1
  IMAPve_g_ESC_UnYawRate_1/1 -> IMAPve_g_ESC_UnYawRate_2/1
  IMAPve_g_ESC_VehSpd/1 -> IMAPve_g_ESC_VehSpd_1/1
  IMAPve_g_ESC_VehSpd_1/1 -> IMAPve_g_ESC_VehSpd_2/1
  IMAPve_g_ESC_LonAcc/1 -> IMAPve_g_ESC_LonAcc_1/1
  IMAPve_g_ESC_LonAcc_1/1 -> IMAPve_g_ESC_LonAcc_2/1
  IMAPve_d_ESC_LonAcc_Valid/1 -> IMAPve_d_ESC_LonAcc_Valid_1/1
  IMAPve_d_ESC_LonAcc_Valid_1/1 -> IMAPve_d_ESC_LonAcc_Valid_2/1
  IMAPve_g_ESC_Brake_Press/1 -> IMAPve_g_ESC_Brake_Press_1/1
  IMAPve_g_ESC_Brake_Press_1/1 -> IMAPve_g_ESC_Brake_Press_2/1
  IMAPve_g_ESC_Static_Slope/1 -> IMAPve_g_ESC_Static_Slope_1/1
  IMAPve_g_ESC_Static_Slope_1/1 -> IMAPve_g_ESC_Static_Slope_2/1
  IMAPve_g_ESC_DySlope_Accuracy/1 -> IMAPve_g_ESC_DySlope_Accuracy_1/1
  IMAPve_g_ESC_DySlope_Accuracy_1/1 -> IMAPve_g_ESC_DySlope_Accuracy_2/1
  IMAPve_g_ESC_DySlope/1 -> IMAPve_g_ESC_DySlope_1/1
  IMAPve_g_ESC_DySlope_1/1 -> IMAPve_g_ESC_DySlope_2/1
  IMAPve_g_SW_Angle/1 -> IMAPve_g_SW_Angle_1/1
  IMAPve_g_SW_Angle_1/1 -> IMAPve_g_SW_Angle_2/1
  IMAPve_g_SW_Angle_Speed/1 -> IMAPve_g_SW_Angle_Speed_1/1
  IMAPve_g_SW_Angle_Speed_1/1 -> IMAPve_g_SW_Angle_Speed_2/1
  IMAPve_d_BCM_HazardLamp/1 -> IMAPve_d_BCM_HazardLamp_1/1
  IMAPve_d_BCM_HazardLamp_1/1 -> IMAPve_d_BCM_HazardLamp_2/1
  IMAPve_d_BCM_Left_Light/1 -> IMAPve_d_BCM_Left_Light_1/1
  IMAPve_d_BCM_Left_Light_1/1 -> IMAPve_d_BCM_Left_Light_2/1
  IMAPve_d_BCM_Right_Light/1 -> IMAPve_d_BCM_Right_Light_1/1
  IMAPve_d_BCM_Right_Light_1/1 -> IMAPve_d_BCM_Right_Light_2/1
  IMAPve_d_ESC_BrakeLamp_Req/1 -> IMAPve_d_ESC_BrakeLamp_Req_1/1
  IMAPve_d_ESC_BrakeLamp_Req_1/1 -> IMAPve_d_ESC_BrakeLamp_Req_2/1
  IMAPve_d_BCM_Opening_State/1 -> IMAPve_d_BCM_Opening_State_1/1
  IMAPve_d_BCM_Opening_State_1/1 -> IMAPve_d_BCM_Opening_State_2/1
  IMAPve_d_BCM_Trunk_State/1 -> IMAPve_d_BCM_Trunk_State_1/1
  IMAPve_d_BCM_Trunk_State_1/1 -> IMAPve_d_BCM_Trunk_State_2/1
  IMAPve_d_BCM_LF_Door_State/1 -> IMAPve_d_BCM_LF_Door_State_1/1
  IMAPve_d_BCM_LF_Door_State_1/1 -> IMAPve_d_BCM_LF_Door_State_2/1
  IMAPve_d_BCM_RF_Door_State/1 -> IMAPve_d_BCM_RF_Door_State_1/1
  IMAPve_d_BCM_RF_Door_State_1/1 -> IMAPve_d_BCM_RF_Door_State_2/1
  IMAPve_d_BCM_RR_Door_State/1 -> IMAPve_d_BCM_RR_Door_State_1/1
  IMAPve_d_BCM_RR_Door_State_1/1 -> IMAPve_d_BCM_RR_Door_State_2/1
  IMAPve_d_BCM_LR_Door_State/1 -> IMAPve_d_BCM_LR_Door_State_1/1
  IMAPve_d_BCM_LR_Door_State_1/1 -> IMAPve_d_BCM_LR_Door_State_2/1
  IMAPve_d_SCC_Left_SwitchSig/1 -> IMAPve_d_SCC_Left_SwitchSig_1/1
  IMAPve_d_SCC_Left_SwitchSig_1/1 -> IMAPve_d_SCC_Left_SwitchSig_2/1
  IMAPve_d_SCC_Right_SwitchSig/1 -> IMAPve_d_SCC_Right_SwitchSig_1/1
  IMAPve_d_SCC_Right_SwitchSig_1/1 -> IMAPve_d_SCC_Right_SwitchSig_2/1
  IMAPve_d_PEPS_Door_Lock_Req/1 -> IMAPve_d_PEPS_Door_Lock_Req_1/1
  IMAPve_d_PEPS_Door_Lock_Req_1/1 -> IMAPve_d_PEPS_Door_Lock_Req_2/1
  IMAPve_d_BCM_Door_Lock_State/1 -> IMAPve_d_BCM_Door_Lock_State_1/1
  IMAPve_d_BCM_Door_Lock_State_1/1 -> IMAPve_d_BCM_Door_Lock_State_2/1
  IMAPve_d_EMS_ACC_Status/1 -> IMAPve_d_EMS_ACC_Status_1/1
  IMAPve_d_EMS_ACC_Status_1/1 -> IMAPve_d_EMS_ACC_Status_2/1
  IMAPve_g_EMS_Pot_WhlT_Max/1 -> IMAPve_g_EMS_Pot_WhlT_Max_1/1
  IMAPve_g_EMS_Pot_WhlT_Max_1/1 -> IMAPve_g_EMS_Pot_WhlT_Max_2/1
  IMAPve_g_EMS_Pot_WhlT_Min/1 -> IMAPve_g_EMS_Pot_WhlT_Min_1/1
  IMAPve_g_EMS_Pot_WhlT_Min_1/1 -> IMAPve_g_EMS_Pot_WhlT_Min_2/1
  IMAPve_g_EMS_RealPedal/1 -> IMAPve_g_EMS_RealPedal_1/1
  IMAPve_g_EMS_RealPedal_1/1 -> IMAPve_g_EMS_RealPedal_2/1
  IMAPve_g_EMS_MaxTWhl/1 -> IMAPve_g_EMS_MaxTWhl_1/1
  IMAPve_g_EMS_MaxTWhl_1/1 -> IMAPve_g_EMS_MaxTWhl_2/1
  IMAPve_g_EMS_MaxTWhl_Offset/1 -> IMAPve_g_EMS_MaxTWhl_Offset_1/1
  IMAPve_g_EMS_MaxTWhl_Offset_1/1 -> IMAPve_g_EMS_MaxTWhl_Offset_2/1
  IMAPve_g_EMS_MinTWhl/1 -> IMAPve_g_EMS_MinTWhl_1/1
  IMAPve_g_EMS_MinTWhl_1/1 -> IMAPve_g_EMS_MinTWhl_2/1
  IMAPve_g_EMS_MinTWhl_Offset/1 -> IMAPve_g_EMS_MinTWhl_Offset_1/1
  IMAPve_g_EMS_MinTWhl_Offset_1/1 -> IMAPve_g_EMS_MinTWhl_Offset_2/1
  IMAPve_g_EMS_Actual_FlwT/1 -> IMAPve_g_EMS_Actual_FlwT_1/1
  IMAPve_g_EMS_Actual_FlwT_1/1 -> IMAPve_g_EMS_Actual_FlwT_2/1
  IMAPve_g_EMS_Actual_IndT/1 -> IMAPve_g_EMS_Actual_IndT_1/1
  IMAPve_g_EMS_Actual_IndT_1/1 -> IMAPve_g_EMS_Actual_IndT_2/1
  IMAPve_g_EMS_Realize_TWhl/1 -> IMAPve_g_EMS_Realize_TWhl_1/1
  IMAPve_g_EMS_Realize_TWhl_1/1 -> IMAPve_g_EMS_Realize_TWhl_2/1
  IMAPve_g_EMS_ACC_VirtualPedal/1 -> IMAPve_g_EMS_ACC_VirtualPedal_1/1
  IMAPve_g_EMS_ACC_VirtualPedal_1/1 -> IMAPve_g_EMS_ACC_VirtualPedal_2/1
  IMAPve_d_EMS_AccPedal_Fault/1 -> IMAPve_d_EMS_AccPedal_Fault_1/1
  IMAPve_d_EMS_AccPedal_Fault_1/1 -> IMAPve_d_EMS_AccPedal_Fault_2/1
  IMAPve_g_EMS_Driver_Torque/1 -> IMAPve_g_EMS_Driver_Torque_1/1
  IMAPve_g_EMS_Driver_Torque_1/1 -> IMAPve_g_EMS_Driver_Torque_2/1
  IMAPve_d_ESC_Brake_Effort/1 -> IMAPve_d_ESC_Brake_Effort_1/1
  IMAPve_d_ESC_Brake_Effort_1/1 -> IMAPve_d_ESC_Brake_Effort_2/1
  IMAPve_g_EMS_Engine_Speed/1 -> IMAPve_g_EMS_Engine_Speed_1/1
  IMAPve_g_EMS_Engine_Speed_1/1 -> IMAPve_g_EMS_Engine_Speed_2/1
  IMAPve_d_ESC_Veh_Standstill/1 -> IMAPve_d_ESC_Veh_Standstill_1/1
  IMAPve_d_ESC_Veh_Standstill_1/1 -> IMAPve_d_ESC_Veh_Standstill_2/1
  IMAPve_d_TCU_Actual_Gear/1 -> IMAPve_d_TCU_Actual_Gear_1/1
  IMAPve_d_TCU_Actual_Gear_1/1 -> IMAPve_d_TCU_Actual_Gear_2/1
  IMAPve_d_TCU_Target_Gear/1 -> IMAPve_d_TCU_Target_Gear_1/1
  IMAPve_d_TCU_Target_Gear_1/1 -> IMAPve_d_TCU_Target_Gear_2/1
  IMAPve_d_TCU_PRND_State/1 -> IMAPve_d_TCU_PRND_State_1/1
  IMAPve_d_TCU_PRND_State_1/1 -> IMAPve_d_TCU_PRND_State_2/1
  IMAPve_d_BCM_Ignition_State/1 -> IMAPve_d_BCM_Ignition_State_1/1
  IMAPve_d_BCM_Ignition_State_1/1 -> IMAPve_d_BCM_Ignition_State_2/1
  IMAPve_d_ACU_Driver_Belt/1 -> IMAPve_d_ACU_Driver_Belt_1/1
  IMAPve_d_ACU_Driver_Belt_1/1 -> IMAPve_d_ACU_Driver_Belt_2/1
  IMAPve_d_SWS_Fault_Code/1 -> IMAPve_d_SWS_Fault_Code_1/1
  IMAPve_d_SWS_Fault_Code_1/1 -> IMAPve_d_SWS_Fault_Code_2/1
  IMAPve_d_SWS_Failure_Status/1 -> IMAPve_d_SWS_Failure_Status_1/1
  IMAPve_d_SWS_Failure_Status_1/1 -> IMAPve_d_SWS_Failure_Status_2/1
  IMAPve_d_ESC_OFF/1 -> IMAPve_d_ESC_OFF_1/1
  IMAPve_d_ESC_OFF_1/1 -> IMAPve_d_ESC_OFF_2/1
  IMAPve_d_ESC_AlarmSig/1 -> IMAPve_d_ESC_AlarmSig_1/1
  IMAPve_d_ESC_AlarmSig_1/1 -> IMAPve_d_ESC_AlarmSig_2/1
  IMAPve_d_Speed_Limit_Switch/1 -> IMAPve_d_Speed_Limit_Switch_1/1
  IMAPve_d_Speed_Limit_Switch_1/1 -> IMAPve_d_Speed_Limit_Switch_2/1
  IMAPve_d_ESC_ESC_Active/1 -> IMAPve_d_ESC_ESC_Active_1/1
  IMAPve_d_ESC_ESC_Active_1/1 -> IMAPve_d_ESC_ESC_Active_2/1
  IMAPve_d_ESC_MSR_Active/1 -> IMAPve_d_ESC_MSR_Active_1/1
  IMAPve_d_ESC_MSR_Active_1/1 -> IMAPve_d_ESC_MSR_Active_2/1
  IMAPve_d_ESC_TCS_Active/1 -> IMAPve_d_ESC_TCS_Active_1/1
  IMAPve_d_ESC_TCS_Active_1/1 -> IMAPve_d_ESC_TCS_Active_2/1
  IMAPve_d_ESC_VehSpd_Valid/1 -> IMAPve_d_ESC_VehSpd_Valid_1/1
  IMAPve_d_ESC_VehSpd_Valid_1/1 -> IMAPve_d_ESC_VehSpd_Valid_2/1
  IMAPve_d_Brake_Pedal_Fault/1 -> IMAPve_d_Brake_Pedal_Fault_1/1
  IMAPve_d_Brake_Pedal_Fault_1/1 -> IMAPve_d_Brake_Pedal_Fault_2/1
  IMAPve_d_ESC_ABS_Active/1 -> IMAPve_d_ESC_ABS_Active_1/1
  IMAPve_d_ESC_ABS_Active_1/1 -> IMAPve_d_ESC_ABS_Active_2/1
  IMAPve_d_ESC_ABS_Valid/1 -> IMAPve_d_ESC_ABS_Valid_1/1
  IMAPve_d_ESC_ABS_Valid_1/1 -> IMAPve_d_ESC_ABS_Valid_2/1
  IMAPve_d_ESC_ABS_AlarmSig/1 -> IMAPve_d_ESC_ABS_AlarmSig_1/1
  IMAPve_d_ESC_ABS_AlarmSig_1/1 -> IMAPve_d_ESC_ABS_AlarmSig_2/1
  IMAPve_d_ESC_FL_WheelPulVal/1 -> IMAPve_d_ESC_FL_WheelPulVal_1/1
  IMAPve_d_ESC_FL_WheelPulVal_1/1 -> IMAPve_d_ESC_FL_WheelPulVal_2/1
  IMAPve_d_ESC_FR_WheelPulVal/1 -> IMAPve_d_ESC_FR_WheelPulVal_1/1
  IMAPve_d_ESC_FR_WheelPulVal_1/1 -> IMAPve_d_ESC_FR_WheelPulVal_2/1
  IMAPve_d_ESC_RL_WheelPulVal/1 -> IMAPve_d_ESC_RL_WheelPulVal_1/1
  IMAPve_d_ESC_RL_WheelPulVal_1/1 -> IMAPve_d_ESC_RL_WheelPulVal_2/1
  IMAPve_d_ESC_RR_WheelPulVal/1 -> IMAPve_d_ESC_RR_WheelPulVal_1/1
  IMAPve_d_ESC_RR_WheelPulVal_1/1 -> IMAPve_d_ESC_RR_WheelPulVal_2/1
  IMAPve_g_ESC_FL_WhlSpd/1 -> IMAPve_g_ESC_FL_WhlSpd_1/1
  IMAPve_g_ESC_FL_WhlSpd_1/1 -> IMAPve_g_ESC_FL_WhlSpd_2/1
  IMAPve_d_ESC_FL_WhlSpd_Fault/1 -> IMAPve_d_ESC_FL_WhlSpd_Fault_1/1
  IMAPve_d_ESC_FL_WhlSpd_Fault_1/1 -> IMAPve_d_ESC_FL_WhlSpd_Fault_2/1
  IMAPve_g_ESC_FR_WhlSpd/1 -> IMAPve_g_ESC_FR_WhlSpd_1/1
  IMAPve_g_ESC_FR_WhlSpd_1/1 -> IMAPve_g_ESC_FR_WhlSpd_2/1
  IMAPve_d_ESC_FR_WhlSpd_Fault/1 -> IMAPve_d_ESC_FR_WhlSpd_Fault_1/1
  IMAPve_d_ESC_FR_WhlSpd_Fault_1/1 -> IMAPve_d_ESC_FR_WhlSpd_Fault_2/1
  IMAPve_g_ESC_RL_WhlSpd/1 -> IMAPve_g_ESC_RL_WhlSpd_1/1
  IMAPve_g_ESC_RL_WhlSpd_1/1 -> IMAPve_g_ESC_RL_WhlSpd_2/1
  IMAPve_d_ESC_RL_WhlSpd_Fault/1 -> IMAPve_d_ESC_RL_WhlSpd_Fault_1/1
  IMAPve_d_ESC_RL_WhlSpd_Fault_1/1 -> IMAPve_d_ESC_RL_WhlSpd_Fault_2/1
  IMAPve_g_ESC_RR_WhlSpd/1 -> IMAPve_g_ESC_RR_WhlSpd_1/1
  IMAPve_g_ESC_RR_WhlSpd_1/1 -> IMAPve_g_ESC_RR_WhlSpd_2/1
  IMAPve_d_ESC_RR_WhlSpd_Fault/1 -> IMAPve_d_ESC_RR_WhlSpd_Fault_1/1
  IMAPve_d_ESC_RR_WhlSpd_Fault_1/1 -> IMAPve_d_ESC_RR_WhlSpd_Fault_2/1
  IMAPve_d_ESC_FL_Wheel_Pulse/1 -> IMAPve_d_ESC_FL_Wheel_Pulse_1/1
  IMAPve_d_ESC_FL_Wheel_Pulse_1/1 -> IMAPve_d_ESC_FL_Wheel_Pulse_2/1
  IMAPve_d_ESC_FR_Wheel_Pulse/1 -> IMAPve_d_ESC_FR_Wheel_Pulse_1/1
  IMAPve_d_ESC_FR_Wheel_Pulse_1/1 -> IMAPve_d_ESC_FR_Wheel_Pulse_2/1
  IMAPve_d_ESC_RL_Wheel_Pulse/1 -> IMAPve_d_ESC_RL_Wheel_Pulse_1/1
  IMAPve_d_ESC_RL_Wheel_Pulse_1/1 -> IMAPve_d_ESC_RL_Wheel_Pulse_2/1
  IMAPve_d_ESC_RR_Wheel_Pulse/1 -> IMAPve_d_ESC_RR_Wheel_Pulse_1/1
  IMAPve_d_ESC_RR_Wheel_Pulse_1/1 -> IMAPve_d_ESC_RR_Wheel_Pulse_2/1
  IMAPve_d_TCU_AT_Failure/1 -> IMAPve_d_TCU_AT_Failure_1/1
  IMAPve_d_TCU_AT_Failure_1/1 -> IMAPve_d_TCU_AT_Failure_2/1
  IMAPve_d_TCU_Shift_Valid/1 -> IMAPve_d_TCU_Shift_Valid_1/1
  IMAPve_d_TCU_Shift_Valid_1/1 -> IMAPve_d_TCU_Shift_Valid_2/1
  IMAPve_d_TCU_DCT_Clutch_State/1 -> IMAPve_d_TCU_DCT_Clutch_State_1/1
  IMAPve_d_TCU_DCT_Clutch_State_1/1 -> IMAPve_d_TCU_DCT_Clutch_State_2/1
  IMAPve_d_TCU_Gear_Engage/1 -> IMAPve_d_TCU_Gear_Engage_1/1
  IMAPve_d_TCU_Gear_Engage_1/1 -> IMAPve_d_TCU_Gear_Engage_2/1
  IMAPve_d_TCU_Select_ATMode/1 -> IMAPve_d_TCU_Select_ATMode_1/1
  IMAPve_d_TCU_Select_ATMode_1/1 -> IMAPve_d_TCU_Select_ATMode_2/1
  IMAPve_d_EMS_Engine_Status/1 -> IMAPve_d_EMS_Engine_Status_1/1
  IMAPve_d_EMS_Engine_Status_1/1 -> IMAPve_d_EMS_Engine_Status_2/1
  IMAPve_d_EMS_Gearbox_CtlAvail/1 -> IMAPve_d_EMS_Gearbox_CtlAvail_1/1
  IMAPve_d_EMS_Gearbox_CtlAvail_1/1 -> IMAPve_d_EMS_Gearbox_CtlAvail_2/1
  IMAPve_d_ESC_Brake_Failsafe/1 -> IMAPve_d_ESC_Brake_Failsafe_1/1
  IMAPve_d_ESC_Brake_Failsafe_1/1 -> IMAPve_d_ESC_Brake_Failsafe_2/1
  IMAPve_d_ESC_AEB_Status/1 -> IMAPve_d_ESC_AEB_Status_1/1
  IMAPve_d_ESC_AEB_Status_1/1 -> IMAPve_d_ESC_AEB_Status_2/1
  IMAPve_d_ESC_AEB_Available/1 -> IMAPve_d_ESC_AEB_Available_1/1
  IMAPve_d_ESC_AEB_Available_1/1 -> IMAPve_d_ESC_AEB_Available_2/1
  IMAPve_d_ESC_AEB_Active/1 -> IMAPve_d_ESC_AEB_Active_1/1
  IMAPve_d_ESC_AEB_Active_1/1 -> IMAPve_d_ESC_AEB_Active_2/1
  IMAPve_d_ESC_ACC_Status/1 -> IMAPve_d_ESC_ACC_Status_1/1
  IMAPve_d_ESC_ACC_Status_1/1 -> IMAPve_d_ESC_ACC_Status_2/1
  IMAPve_d_ESC_ACC_Available/1 -> IMAPve_d_ESC_ACC_Available_1/1
  IMAPve_d_ESC_ACC_Available_1/1 -> IMAPve_d_ESC_ACC_Available_2/1
  IMAPve_d_ESC_ACC_Active/1 -> IMAPve_d_ESC_ACC_Active_1/1
  IMAPve_d_ESC_ACC_Active_1/1 -> IMAPve_d_ESC_ACC_Active_2/1
  IMAPve_d_EMS_ACC_Effective/1 -> IMAPve_d_EMS_ACC_Effective_1/1
  IMAPve_d_EMS_ACC_Effective_1/1 -> IMAPve_d_EMS_ACC_Effective_2/1
  IMAPve_d_BCM_FrontWiper_State/1 -> IMAPve_d_BCM_FrontWiper_State_1/1
  IMAPve_d_BCM_FrontWiper_State_1/1 -> IMAPve_d_BCM_FrontWiper_State_2/1
  IMAPve_d_BCM_CHMSL_Status/1 -> IMAPve_d_BCM_CHMSL_Status_1/1
  IMAPve_d_BCM_CHMSL_Status_1/1 -> IMAPve_d_BCM_CHMSL_Status_2/1
  IMAPve_d_BCM_BrakeLamp_State/1 -> IMAPve_d_BCM_BrakeLamp_State_1/1
  IMAPve_d_BCM_BrakeLamp_State_1/1 -> IMAPve_d_BCM_BrakeLamp_State_2/1
  IMAPve_d_GW_Brake_Only_Req/1 -> IMAPve_d_GW_Brake_Only_Req_1/1
  IMAPve_d_GW_Brake_Only_Req_1/1 -> IMAPve_d_GW_Brake_Only_Req_2/1
  IMAPve_d_ACU_Passenger_Belt/1 -> IMAPve_d_ACU_Passenger_Belt_1/1
  IMAPve_d_ACU_Passenger_Belt_1/1 -> IMAPve_d_ACU_Passenger_Belt_2/1
  IMAPve_d_EMS_ACC_CtlAvail/1 -> IMAPve_d_EMS_ACC_CtlAvail_1/1
  IMAPve_d_EMS_ACC_CtlAvail_1/1 -> IMAPve_d_EMS_ACC_CtlAvail_2/1
  IMAPve_d_EMS_ACC_Inhibited/1 -> IMAPve_d_EMS_ACC_Inhibited_1/1
  IMAPve_d_EMS_ACC_Inhibited_1/1 -> IMAPve_d_EMS_ACC_Inhibited_2/1
  IMAPve_d_EMS_Brake_Pedal/1 -> IMAPve_d_EMS_Brake_Pedal_1/1
  IMAPve_d_EMS_Brake_Pedal_1/1 -> IMAPve_d_EMS_Brake_Pedal_2/1
  IMAPve_d_BCM_LowBeam_State/1 -> IMAPve_d_BCM_LowBeam_State_1/1
  IMAPve_d_BCM_LowBeam_State_1/1 -> IMAPve_d_BCM_LowBeam_State_2/1
  IMAPve_d_BCM_HighBeam_State/1 -> IMAPve_d_BCM_HighBeam_State_1/1
  IMAPve_d_BCM_HighBeam_State_1/1 -> IMAPve_d_BCM_HighBeam_State_2/1
  IMAPve_d_EPB_Status/1 -> IMAPve_d_EPB_Status_1/1
  IMAPve_d_EPB_Status_1/1 -> IMAPve_d_EPB_Status_2/1
  IMAPve_d_EPB_Display_Req/1 -> IMAPve_d_EPB_Display_Req_1/1
  IMAPve_d_EPB_Display_Req_1/1 -> IMAPve_d_EPB_Display_Req_2/1
  IMAPve_d_EPB_Warn_Req/1 -> IMAPve_d_EPB_Warn_Req_1/1
  IMAPve_d_EPB_Warn_Req_1/1 -> IMAPve_d_EPB_Warn_Req_2/1
  IMAPve_d_EPB_Switch_State/1 -> IMAPve_d_EPB_Switch_State_1/1
  IMAPve_d_EPB_Switch_State_1/1 -> IMAPve_d_EPB_Switch_State_2/1
  IMAPve_d_EPB_Switch_Valid/1 -> IMAPve_d_EPB_Switch_Valid_1/1
  IMAPve_d_EPB_Switch_Valid_1/1 -> IMAPve_d_EPB_Switch_Valid_2/1
  IMAPve_d_ESC_Drive_Direction/1 -> IMAPve_d_ESC_Drive_Direction_1/1
  IMAPve_d_ESC_Drive_Direction_1/1 -> IMAPve_d_ESC_Drive_Direction_2/1
  IMAPve_d_ESC_Hold_State/1 -> IMAPve_d_ESC_Hold_State_1/1
  IMAPve_d_ESC_Hold_State_1/1 -> IMAPve_d_ESC_Hold_State_2/1
  IMAPve_d_EPS_Steer_Hold_State/1 -> IMAPve_d_EPS_Steer_Hold_State_1/1
  IMAPve_d_EPS_Steer_Hold_State_1/1 -> IMAPve_d_EPS_Steer_Hold_State_2/1
  IMAPve_d_EPS_Warning_State/1 -> IMAPve_d_EPS_Warning_State_1/1
  IMAPve_d_EPS_Warning_State_1/1 -> IMAPve_d_EPS_Warning_State_2/1
  IMAPve_g_EPS_PowerCon/1 -> IMAPve_g_EPS_PowerCon_1/1
  IMAPve_g_EPS_PowerCon_1/1 -> IMAPve_g_EPS_PowerCon_2/1
  IMAPve_d_ESC_EBD_AlarmSig/1 -> IMAPve_d_ESC_EBD_AlarmSig_1/1
  IMAPve_d_ESC_EBD_AlarmSig_1/1 -> IMAPve_d_ESC_EBD_AlarmSig_2/1
  IMAPve_d_ESC_AVH_Status/1 -> IMAPve_d_ESC_AVH_Status_1/1
  IMAPve_d_ESC_AVH_Status_1/1 -> IMAPve_d_ESC_AVH_Status_2/1
  IMAPve_d_Radar_Detective_Req/1 -> IMAPve_d_Radar_Detective_Req_1/1
  IMAPve_d_Radar_Detective_Req_1/1 -> IMAPve_d_Radar_Detective_Req_2/1
  IMAPve_g_BCM_Battery_Voltage/1 -> IMAPve_g_BCM_Battery_Voltage_1/1
  IMAPve_g_BCM_Battery_Voltage_1/1 -> IMAPve_g_BCM_Battery_Voltage_2/1
  IMAPve_d_TBOX_LocalTimeY/1 -> IMAPve_d_TBOX_LocalTimeY_1/1
  IMAPve_d_TBOX_LocalTimeY_1/1 -> IMAPve_d_TBOX_LocalTimeY_2/1
  IMAPve_d_TBOX_LocalTimeM/1 -> IMAPve_d_TBOX_LocalTimeM_1/1
  IMAPve_d_TBOX_LocalTimeM_1/1 -> IMAPve_d_TBOX_LocalTimeM_2/1
  IMAPve_d_TBOX_LocalTimeD/1 -> IMAPve_d_TBOX_LocalTimeD_1/1
  IMAPve_d_TBOX_LocalTimeD_1/1 -> IMAPve_d_TBOX_LocalTimeD_2/1
  IMAPve_d_TBOX_LocalTimeH/1 -> IMAPve_d_TBOX_LocalTimeH_1/1
  IMAPve_d_TBOX_LocalTimeH_1/1 -> IMAPve_d_TBOX_LocalTimeH_2/1
  IMAPve_d_TBOX_LocalTimeMin/1 -> IMAPve_d_TBOX_LocalTimeMin_1/1
  IMAPve_d_TBOX_LocalTimeMin_1/1 -> IMAPve_d_TBOX_LocalTimeMin_2/1
  IMAPve_d_TBOX_LocalTimeS/1 -> IMAPve_d_TBOX_LocalTimeS_1/1
  IMAPve_d_TBOX_LocalTimeS_1/1 -> IMAPve_d_TBOX_LocalTimeS_2/1
  IMAPve_d_TBOX_LocalTime_Valid/1 -> IMAPve_d_TBOX_LocalTime_Valid_1/1
  IMAPve_d_TBOX_LocalTime_Valid_1/1 -> IMAPve_d_TBOX_LocalTime_Valid_2/1
  IMAPve_d_TPMS_Warn_Indicate/1 -> IMAPve_d_TPMS_Warn_Indicate_1/1
  IMAPve_d_TPMS_Warn_Indicate_1/1 -> IMAPve_d_TPMS_Warn_Indicate_2/1
  IMAPve_d_Radar_State/1 -> IMAPve_d_Radar_State_1/1
  IMAPve_d_Radar_State_1/1 -> IMAPve_d_Radar_State_2/1
  IMAPve_d_ACC_Desired_Headway/1 -> IMAPve_d_ACC_Desired_Headway_1/1
  IMAPve_d_ACC_Desired_Headway_1/1 -> IMAPve_d_ACC_Desired_Headway_2/1
  IMAPve_d_Time_System_Clock/1 -> IMAPve_d_Time_System_Clock_1/1
  IMAPve_d_Time_System_Clock_1/1 -> IMAPve_d_Time_System_Clock_2/1
  IMAPve_d_Signal_Time_Stamp/1 -> IMAPve_d_Signal_Time_Stamp_1/1
  IMAPve_d_Signal_Time_Stamp_1/1 -> IMAPve_d_Signal_Time_Stamp_2/1
  IMAPve_g_GW_IC_Odometer/1 -> IMAPve_g_GW_IC_Odometer_1/1
  IMAPve_g_GW_IC_Odometer_1/1 -> IMAPve_g_GW_IC_Odometer_2/1
  IMAPve_g_FAPA_State/1 -> IMAPve_g_FAPA_State_1/1
  IMAPve_g_FAPA_State_1/1 -> IMAPve_g_FAPA_State_2/1
  IMAPve_d_Outside_Temp/1 -> IMAPve_d_Outside_Temp_1/1
  IMAPve_d_Outside_Temp_1/1 -> IMAPve_d_Outside_Temp_2/1
  IMAPve_d_ORI_CIPV_ID/1 -> IMAPve_d_ORI_CIPV_ID_1/1
  IMAPve_d_ORI_CIPV_ID_1/1 -> IMAPve_d_ORI_CIPV_ID_2/1
  IMAPve_d_ORI_Obj_Num/1 -> IMAPve_d_ORI_Obj_Num_1/1
  IMAPve_d_ORI_Obj_Num_1/1 -> IMAPve_d_ORI_Obj_Num_2/1
  IMAPva_g_ORI_Probability/1 -> IMAPva_g_ORI_Probability_1/1
  IMAPva_g_ORI_Probability_1/1 -> IMAPva_g_ORI_Probability_2/1
  IMAPva_d_ORI_Obj_Class/1 -> IMAPva_d_ORI_Obj_Class_1/1
  IMAPva_d_ORI_Obj_Class_1/1 -> IMAPva_d_ORI_Obj_Class_2/1
  IMAPva_d_ORI_Obj_Motion/1 -> IMAPva_d_ORI_Obj_Motion_1/1
  IMAPva_d_ORI_Obj_Motion_1/1 -> IMAPva_d_ORI_Obj_Motion_2/1
  IMAPva_g_ORI_Obj_RelVel/1 -> IMAPva_g_ORI_Obj_RelVel_1/1
  IMAPva_g_ORI_Obj_RelVel_1/1 -> IMAPva_g_ORI_Obj_RelVel_2/1
  IMAPva_g_ORI_Obj_LongDis/1 -> IMAPva_g_ORI_Obj_LongDis_1/1
  IMAPva_g_ORI_Obj_LongDis_1/1 -> IMAPva_g_ORI_Obj_LongDis_2/1
  IMAPva_d_ORI_Obj_Lane/1 -> IMAPva_d_ORI_Obj_Lane_1/1
  IMAPva_d_ORI_Obj_Lane_1/1 -> IMAPva_d_ORI_Obj_Lane_2/1
  IMAPva_g_ORI_Obj_LAngle/1 -> IMAPva_g_ORI_Obj_LAngle_1/1
  IMAPva_g_ORI_Obj_LAngle_1/1 -> IMAPva_g_ORI_Obj_LAngle_2/1
  IMAPva_g_ORI_Obj_RAngle/1 -> IMAPva_g_ORI_Obj_RAngle_1/1
  IMAPva_g_ORI_Obj_RAngle_1/1 -> IMAPva_g_ORI_Obj_RAngle_2/1
  IMAPva_g_ORI_Obj_Width/1 -> IMAPva_g_ORI_Obj_Width_1/1
  IMAPva_g_ORI_Obj_Width_1/1 -> IMAPva_g_ORI_Obj_Width_2/1
  IMAPva_d_ORI_Obj_ID/1 -> IMAPva_d_ORI_Obj_ID_1/1
  IMAPva_d_ORI_Obj_ID_1/1 -> IMAPva_d_ORI_Obj_ID_2/1
  IMAPve_d_ORI_Lane_Valid/1 -> IMAPve_d_ORI_Lane_Valid_1/1
  IMAPve_d_ORI_Lane_Valid_1/1 -> IMAPve_d_ORI_Lane_Valid_2/1
  IMAPve_d_ORI_Lane_ConsArea/1 -> IMAPve_d_ORI_Lane_ConsArea_1/1
  IMAPve_d_ORI_Lane_ConsArea_1/1 -> IMAPve_d_ORI_Lane_ConsArea_2/1
  IMAPve_d_ORI_Lane_RoadType/1 -> IMAPve_d_ORI_Lane_RoadType_1/1
  IMAPve_d_ORI_Lane_RoadType_1/1 -> IMAPve_d_ORI_Lane_RoadType_2/1
  IMAPve_g_ORI_L0_C3/1 -> IMAPve_g_ORI_L0_C3_1/1
  IMAPve_g_ORI_L0_C3_1/1 -> IMAPve_g_ORI_L0_C3_2/1
  IMAPve_g_ORI_L0_C2/1 -> IMAPve_g_ORI_L0_C2_1/1
  IMAPve_g_ORI_L0_C2_1/1 -> IMAPve_g_ORI_L0_C2_2/1
  IMAPve_g_ORI_L0_C1/1 -> IMAPve_g_ORI_L0_C1_1/1
  IMAPve_g_ORI_L0_C1_1/1 -> IMAPve_g_ORI_L0_C1_2/1
  IMAPve_g_ORI_L0_C0/1 -> IMAPve_g_ORI_L0_C0_1/1
  IMAPve_g_ORI_L0_C0_1/1 -> IMAPve_g_ORI_L0_C0_2/1
  IMAPve_d_ORI_L0_Q/1 -> IMAPve_d_ORI_L0_Q_1/1
  IMAPve_d_ORI_L0_Q_1/1 -> IMAPve_d_ORI_L0_Q_2/1
  IMAPve_d_ORI_L0_Type/1 -> IMAPve_d_ORI_L0_Type_1/1
  IMAPve_d_ORI_L0_Type_1/1 -> IMAPve_d_ORI_L0_Type_2/1
  IMAPve_g_ORI_L0_VR/1 -> IMAPve_g_ORI_L0_VR_1/1
  IMAPve_g_ORI_L0_VR_1/1 -> IMAPve_g_ORI_L0_VR_2/1
  IMAPve_g_ORI_L0_TLC/1 -> IMAPve_g_ORI_L0_TLC_1/1
  IMAPve_g_ORI_L0_TLC_1/1 -> IMAPve_g_ORI_L0_TLC_2/1
  IMAPve_g_ORI_L0_W/1 -> IMAPve_g_ORI_L0_W_1/1
  IMAPve_g_ORI_L0_W_1/1 -> IMAPve_g_ORI_L0_W_2/1
  IMAPve_d_ORI_L0_LC/1 -> IMAPve_d_ORI_L0_LC_1/1
  IMAPve_d_ORI_L0_LC_1/1 -> IMAPve_d_ORI_L0_LC_2/1
  IMAPve_g_ORI_L1_C3/1 -> IMAPve_g_ORI_L1_C3_1/1
  IMAPve_g_ORI_L1_C3_1/1 -> IMAPve_g_ORI_L1_C3_2/1
  IMAPve_g_ORI_L1_C2/1 -> IMAPve_g_ORI_L1_C2_1/1
  IMAPve_g_ORI_L1_C2_1/1 -> IMAPve_g_ORI_L1_C2_2/1
  IMAPve_g_ORI_L1_C1/1 -> IMAPve_g_ORI_L1_C1_1/1
  IMAPve_g_ORI_L1_C1_1/1 -> IMAPve_g_ORI_L1_C1_2/1
  IMAPve_g_ORI_L1_C0/1 -> IMAPve_g_ORI_L1_C0_1/1
  IMAPve_g_ORI_L1_C0_1/1 -> IMAPve_g_ORI_L1_C0_2/1
  IMAPve_d_ORI_L1_Q/1 -> IMAPve_d_ORI_L1_Q_1/1
  IMAPve_d_ORI_L1_Q_1/1 -> IMAPve_d_ORI_L1_Q_2/1
  IMAPve_d_ORI_L1_Type/1 -> IMAPve_d_ORI_L1_Type_1/1
  IMAPve_d_ORI_L1_Type_1/1 -> IMAPve_d_ORI_L1_Type_2/1
  IMAPve_g_ORI_L1_VR/1 -> IMAPve_g_ORI_L1_VR_1/1
  IMAPve_g_ORI_L1_VR_1/1 -> IMAPve_g_ORI_L1_VR_2/1
  IMAPve_g_ORI_L1_TLC/1 -> IMAPve_g_ORI_L1_TLC_1/1
  IMAPve_g_ORI_L1_TLC_1/1 -> IMAPve_g_ORI_L1_TLC_2/1
  IMAPve_g_ORI_L1_W/1 -> IMAPve_g_ORI_L1_W_1/1
  IMAPve_g_ORI_L1_W_1/1 -> IMAPve_g_ORI_L1_W_2/1
  IMAPve_d_ORI_L1_LC/1 -> IMAPve_d_ORI_L1_LC_1/1
  IMAPve_d_ORI_L1_LC_1/1 -> IMAPve_d_ORI_L1_LC_2/1
  IMAPve_g_ORI_R0_C3/1 -> IMAPve_g_ORI_R0_C3_1/1
  IMAPve_g_ORI_R0_C3_1/1 -> IMAPve_g_ORI_R0_C3_2/1
  IMAPve_g_ORI_R0_C2/1 -> IMAPve_g_ORI_R0_C2_1/1
  IMAPve_g_ORI_R0_C2_1/1 -> IMAPve_g_ORI_R0_C2_2/1
  IMAPve_g_ORI_R0_C1/1 -> IMAPve_g_ORI_R0_C1_1/1
  IMAPve_g_ORI_R0_C1_1/1 -> IMAPve_g_ORI_R0_C1_2/1
  IMAPve_g_ORI_R0_C0/1 -> IMAPve_g_ORI_R0_C0_1/1
  IMAPve_g_ORI_R0_C0_1/1 -> IMAPve_g_ORI_R0_C0_2/1
  IMAPve_d_ORI_R0_Q/1 -> IMAPve_d_ORI_R0_Q_1/1
  IMAPve_d_ORI_R0_Q_1/1 -> IMAPve_d_ORI_R0_Q_2/1
  IMAPve_d_ORI_R0_LT/1 -> IMAPve_d_ORI_R0_LT_1/1
  IMAPve_d_ORI_R0_LT_1/1 -> IMAPve_d_ORI_R0_LT_2/1
  IMAPve_g_ORI_R0_VR/1 -> IMAPve_g_ORI_R0_VR_1/1
  IMAPve_g_ORI_R0_VR_1/1 -> IMAPve_g_ORI_R0_VR_2/1
  IMAPve_g_ORI_R0_TLC/1 -> IMAPve_g_ORI_R0_TLC_1/1
  IMAPve_g_ORI_R0_TLC_1/1 -> IMAPve_g_ORI_R0_TLC_2/1
  IMAPve_g_ORI_R0_W/1 -> IMAPve_g_ORI_R0_W_1/1
  IMAPve_g_ORI_R0_W_1/1 -> IMAPve_g_ORI_R0_W_2/1
  IMAPve_d_ORI_R0_LC/1 -> IMAPve_d_ORI_R0_LC_1/1
  IMAPve_d_ORI_R0_LC_1/1 -> IMAPve_d_ORI_R0_LC_2/1
  IMAPve_g_ORI_R1_C3/1 -> IMAPve_g_ORI_R1_C3_1/1
  IMAPve_g_ORI_R1_C3_1/1 -> IMAPve_g_ORI_R1_C3_2/1
  IMAPve_g_ORI_R1_C2/1 -> IMAPve_g_ORI_R1_C2_1/1
  IMAPve_g_ORI_R1_C2_1/1 -> IMAPve_g_ORI_R1_C2_2/1
  IMAPve_g_ORI_R1_C1/1 -> IMAPve_g_ORI_R1_C1_1/1
  IMAPve_g_ORI_R1_C1_1/1 -> IMAPve_g_ORI_R1_C1_2/1
  IMAPve_g_ORI_R1_C0/1 -> IMAPve_g_ORI_R1_C0_1/1
  IMAPve_g_ORI_R1_C0_1/1 -> IMAPve_g_ORI_R1_C0_2/1
  IMAPve_d_ORI_R1_Q/1 -> IMAPve_d_ORI_R1_Q_1/1
  IMAPve_d_ORI_R1_Q_1/1 -> IMAPve_d_ORI_R1_Q_2/1
  IMAPve_d_ORI_R1_LT/1 -> IMAPve_d_ORI_R1_LT_1/1
  IMAPve_d_ORI_R1_LT_1/1 -> IMAPve_d_ORI_R1_LT_2/1
  IMAPve_g_ORI_R1_VR/1 -> IMAPve_g_ORI_R1_VR_1/1
  IMAPve_g_ORI_R1_VR_1/1 -> IMAPve_g_ORI_R1_VR_2/1
  IMAPve_g_ORI_R1_TLC/1 -> IMAPve_g_ORI_R1_TLC_1/1
  IMAPve_g_ORI_R1_TLC_1/1 -> IMAPve_g_ORI_R1_TLC_2/1
  IMAPve_g_ORI_R1_W/1 -> IMAPve_g_ORI_R1_W_1/1
  IMAPve_g_ORI_R1_W_1/1 -> IMAPve_g_ORI_R1_W_2/1
  IMAPve_d_ORI_R1_LC/1 -> IMAPve_d_ORI_R1_LC_1/1
  IMAPve_d_ORI_R1_LC_1/1 -> IMAPve_d_ORI_R1_LC_2/1
  IMAPve_d_Sensor_Status/1 -> IMAPve_d_Sensor_Status_1/1
  IMAPve_d_Sensor_Status_1/1 -> IMAPve_d_Sensor_Status_2/1
  IMAPve_d_LF_Radar_Status/1 -> IMAPve_d_LF_Radar_Status_1/1
  IMAPve_d_LF_Radar_Status_1/1 -> IMAPve_d_LF_Radar_Status_2/1
  IMAPve_d_RF_Radar_Status/1 -> IMAPve_d_RF_Radar_Status_1/1
  IMAPve_d_RF_Radar_Status_1/1 -> IMAPve_d_RF_Radar_Status_2/1
  IMAPve_d_LR_Radar_Status/1 -> IMAPve_d_LR_Radar_Status_1/1
  IMAPve_d_LR_Radar_Status_1/1 -> IMAPve_d_LR_Radar_Status_2/1
  IMAPve_d_RR_Radar_Status/1 -> IMAPve_d_RR_Radar_Status_1/1
  IMAPve_d_RR_Radar_Status_1/1 -> IMAPve_d_RR_Radar_Status_2/1
  IMAPve_d_Fusion_Status/1 -> IMAPve_d_Fusion_Status_1/1
  IMAPve_d_Fusion_Status_1/1 -> IMAPve_d_Fusion_Status_2/1
  IMAPve_g_Fusion_Time_Stamp/1 -> IMAPve_g_Fusion_Time_Stamp_1/1
  IMAPve_g_Fusion_Time_Stamp_1/1 -> IMAPve_g_Fusion_Time_Stamp_2/1
  IMAPve_d_obj_Num/1 -> IMAPve_d_obj_Num_1/1
  IMAPve_d_obj_Num_1/1 -> IMAPve_d_obj_Num_2/1
  IMAPva_d_obj_id/1 -> IMAPva_d_obj_id_1/1
  IMAPva_d_obj_id_1/1 -> IMAPva_d_obj_id_2/1
  IMAPva_g_obj_pos_x/1 -> IMAPva_g_obj_pos_x_1/1
  IMAPva_g_obj_pos_x_1/1 -> IMAPva_g_obj_pos_x_2/1
  IMAPva_g_obj_pos_y/1 -> IMAPva_g_obj_pos_y_1/1
  IMAPva_g_obj_pos_y_1/1 -> IMAPva_g_obj_pos_y_2/1
  IMAPva_g_obj_vel_x/1 -> IMAPva_g_obj_vel_x_1/1
  IMAPva_g_obj_vel_x_1/1 -> IMAPva_g_obj_vel_x_2/1
  IMAPva_g_obj_vel_y/1 -> IMAPva_g_obj_vel_y_1/1
  IMAPva_g_obj_vel_y_1/1 -> IMAPva_g_obj_vel_y_2/1
  IMAPva_g_obj_acc_x/1 -> IMAPva_g_obj_acc_x_1/1
  IMAPva_g_obj_acc_x_1/1 -> IMAPva_g_obj_acc_x_2/1
  IMAPva_g_obj_acc_y/1 -> IMAPva_g_obj_acc_y_1/1
  IMAPva_g_obj_acc_y_1/1 -> IMAPva_g_obj_acc_y_2/1
  IMAPva_g_obj_pos_var_x/1 -> IMAPva_g_obj_pos_var_x_1/1
  IMAPva_g_obj_pos_var_x_1/1 -> IMAPva_g_obj_pos_var_x_2/1
  IMAPva_g_obj_pos_var_y/1 -> IMAPva_g_obj_pos_var_y_1/1
  IMAPva_g_obj_pos_var_y_1/1 -> IMAPva_g_obj_pos_var_y_2/1
  IMAPva_g_obj_pos_var_xy/1 -> IMAPva_g_obj_pos_var_xy_1/1
  IMAPva_g_obj_pos_var_xy_1/1 -> IMAPva_g_obj_pos_var_xy_2/1
  IMAPva_g_obj_vel_var_x/1 -> IMAPva_g_obj_vel_var_x_1/1
  IMAPva_g_obj_vel_var_x_1/1 -> IMAPva_g_obj_vel_var_x_2/1
  IMAPva_g_obj_vel_var_y/1 -> IMAPva_g_obj_vel_var_y_1/1
  IMAPva_g_obj_vel_var_y_1/1 -> IMAPva_g_obj_vel_var_y_2/1
  IMAPva_g_obj_vel_var_xy/1 -> IMAPva_g_obj_vel_var_xy_1/1
  IMAPva_g_obj_vel_var_xy_1/1 -> IMAPva_g_obj_vel_var_xy_2/1
  IMAPva_g_obj_width/1 -> IMAPva_g_obj_width_1/1
  IMAPva_g_obj_width_1/1 -> IMAPva_g_obj_width_2/1
  IMAPva_g_obj_length/1 -> IMAPva_g_obj_length_1/1
  IMAPva_g_obj_length_1/1 -> IMAPva_g_obj_length_2/1
  IMAPva_d_obj_fusion_type/1 -> IMAPva_d_obj_fusion_type_1/1
  IMAPva_d_obj_fusion_type_1/1 -> IMAPva_d_obj_fusion_type_2/1
  IMAPva_d_obj_class/1 -> IMAPva_d_obj_class_1/1
  IMAPva_d_obj_class_1/1 -> IMAPva_d_obj_class_2/1
  IMAPva_d_obj_lane/1 -> IMAPva_d_obj_lane_1/1
  IMAPva_d_obj_lane_1/1 -> IMAPva_d_obj_lane_2/1
  IMAPva_d_obj_status/1 -> IMAPva_d_obj_status_1/1
  IMAPva_d_obj_status_1/1 -> IMAPva_d_obj_status_2/1
  IMAPva_d_obj_cam_asso_id/1 -> IMAPva_d_obj_cam_asso_id_1/1
  IMAPva_d_obj_cam_asso_id_1/1 -> IMAPva_d_obj_cam_asso_id_2/1
  IMAPva_g_obj_con/1 -> IMAPva_g_obj_con_1/1
  IMAPva_g_obj_con_1/1 -> IMAPva_g_obj_con_2/1
  IMAPva_g_obj_age/1 -> IMAPva_g_obj_age_1/1
  IMAPva_g_obj_age_1/1 -> IMAPva_g_obj_age_2/1
  IMAPva_d_obj_TurnLight/1 -> IMAPva_d_obj_TurnLight_1/1
  IMAPva_d_obj_TurnLight_1/1 -> IMAPva_d_obj_TurnLight_2/1
  IMAPva_d_obj_BrakeLight/1 -> IMAPva_d_obj_BrakeLight_1/1
  IMAPva_d_obj_BrakeLight_1/1 -> IMAPva_d_obj_BrakeLight_2/1
  IMAPva_d_obj_MotionStatus/1 -> IMAPva_d_obj_MotionStatus_1/1
  IMAPva_d_obj_MotionStatus_1/1 -> IMAPva_d_obj_MotionStatus_2/1
  IMAPva_d_obj_ACC/1 -> IMAPva_d_obj_ACC_1/1
  IMAPva_d_obj_ACC_1/1 -> IMAPva_d_obj_ACC_2/1
  IMAPva_d_obj_AEB/1 -> IMAPva_d_obj_AEB_1/1
  IMAPva_d_obj_AEB_1/1 -> IMAPva_d_obj_AEB_2/1
  IMAPva_d_obj_ELK/1 -> IMAPva_d_obj_ELK_1/1
  IMAPva_d_obj_ELK_1/1 -> IMAPva_d_obj_ELK_2/1
  IMAPva_d_obj_ALC/1 -> IMAPva_d_obj_ALC_1/1
  IMAPva_d_obj_ALC_1/1 -> IMAPva_d_obj_ALC_2/1
  IMAPva_d_obj_ESA/1 -> IMAPva_d_obj_ESA_1/1
  IMAPva_d_obj_ESA_1/1 -> IMAPva_d_obj_ESA_2/1
  IMAPva_d_obj_JA/1 -> IMAPva_d_obj_JA_1/1
  IMAPva_d_obj_JA_1/1 -> IMAPva_d_obj_JA_2/1
  IMAPve_d_Lane_Valid/1 -> IMAPve_d_Lane_Valid_1/1
  IMAPve_d_Lane_Valid_1/1 -> IMAPve_d_Lane_Valid_2/1
  IMAPve_d_Road_Type/1 -> IMAPve_d_Road_Type_1/1
  IMAPve_d_Road_Type_1/1 -> IMAPve_d_Road_Type_2/1
  IMAPve_d_ConsArea/1 -> IMAPve_d_ConsArea_1/1
  IMAPve_d_ConsArea_1/1 -> IMAPve_d_ConsArea_2/1
  IMAPve_g_L0_C0/1 -> IMAPve_g_L0_C0_1/1
  IMAPve_g_L0_C0_1/1 -> IMAPve_g_L0_C0_2/1
  IMAPve_g_L0_C1/1 -> IMAPve_g_L0_C1_1/1
  IMAPve_g_L0_C1_1/1 -> IMAPve_g_L0_C1_2/1
  IMAPve_g_L0_C2/1 -> IMAPve_g_L0_C2_1/1
  IMAPve_g_L0_C2_1/1 -> IMAPve_g_L0_C2_2/1
  IMAPve_g_L0_C3/1 -> IMAPve_g_L0_C3_1/1
  IMAPve_g_L0_C3_1/1 -> IMAPve_g_L0_C3_2/1
  IMAPve_g_L0_VR/1 -> IMAPve_g_L0_VR_1/1
  IMAPve_g_L0_VR_1/1 -> IMAPve_g_L0_VR_2/1
  IMAPve_d_L0_Q/1 -> IMAPve_d_L0_Q_1/1
  IMAPve_d_L0_Q_1/1 -> IMAPve_d_L0_Q_2/1
  IMAPve_d_L0_Type/1 -> IMAPve_d_L0_Type_1/1
  IMAPve_d_L0_Type_1/1 -> IMAPve_d_L0_Type_2/1
  IMAPve_g_L0_Confidence/1 -> IMAPve_g_L0_Confidence_1/1
  IMAPve_g_L0_Confidence_1/1 -> IMAPve_g_L0_Confidence_2/1
  IMAPve_g_L0_W/1 -> IMAPve_g_L0_W_1/1
  IMAPve_g_L0_W_1/1 -> IMAPve_g_L0_W_2/1
  IMAPve_g_L0_TLC/1 -> IMAPve_g_L0_TLC_1/1
  IMAPve_g_L0_TLC_1/1 -> IMAPve_g_L0_TLC_2/1
  IMAPve_d_L0_LC/1 -> IMAPve_d_L0_LC_1/1
  IMAPve_d_L0_LC_1/1 -> IMAPve_d_L0_LC_2/1
  IMAPve_g_R0_C0/1 -> IMAPve_g_R0_C0_1/1
  IMAPve_g_R0_C0_1/1 -> IMAPve_g_R0_C0_2/1
  IMAPve_g_R0_C1/1 -> IMAPve_g_R0_C1_1/1
  IMAPve_g_R0_C1_1/1 -> IMAPve_g_R0_C1_2/1
  IMAPve_g_R0_C2/1 -> IMAPve_g_R0_C2_1/1
  IMAPve_g_R0_C2_1/1 -> IMAPve_g_R0_C2_2/1
  IMAPve_g_R0_C3/1 -> IMAPve_g_R0_C3_1/1
  IMAPve_g_R0_C3_1/1 -> IMAPve_g_R0_C3_2/1
  IMAPve_g_R0_VR/1 -> IMAPve_g_R0_VR_1/1
  IMAPve_g_R0_VR_1/1 -> IMAPve_g_R0_VR_2/1
  IMAPve_d_R0_Q/1 -> IMAPve_d_R0_Q_1/1
  IMAPve_d_R0_Q_1/1 -> IMAPve_d_R0_Q_2/1
  IMAPve_d_R0_Type/1 -> IMAPve_d_R0_Type_1/1
  IMAPve_d_R0_Type_1/1 -> IMAPve_d_R0_Type_2/1
  IMAPve_g_R0_Confidence/1 -> IMAPve_g_R0_Confidence_1/1
  IMAPve_g_R0_Confidence_1/1 -> IMAPve_g_R0_Confidence_2/1
  IMAPve_g_R0_W/1 -> IMAPve_g_R0_W_1/1
  IMAPve_g_R0_W_1/1 -> IMAPve_g_R0_W_2/1
  IMAPve_g_R0_TLC/1 -> IMAPve_g_R0_TLC_1/1
  IMAPve_g_R0_TLC_1/1 -> IMAPve_g_R0_TLC_2/1
  IMAPve_d_R0_LC/1 -> IMAPve_d_R0_LC_1/1
  IMAPve_d_R0_LC_1/1 -> IMAPve_d_R0_LC_2/1
  IMAPve_g_L1_C0/1 -> IMAPve_g_L1_C0_1/1
  IMAPve_g_L1_C0_1/1 -> IMAPve_g_L1_C0_2/1
  IMAPve_g_L1_C1/1 -> IMAPve_g_L1_C1_1/1
  IMAPve_g_L1_C1_1/1 -> IMAPve_g_L1_C1_2/1
  IMAPve_g_L1_C2/1 -> IMAPve_g_L1_C2_1/1
  IMAPve_g_L1_C2_1/1 -> IMAPve_g_L1_C2_2/1
  IMAPve_g_L1_C3/1 -> IMAPve_g_L1_C3_1/1
  IMAPve_g_L1_C3_1/1 -> IMAPve_g_L1_C3_2/1
  IMAPve_g_L1_VR/1 -> IMAPve_g_L1_VR_1/1
  IMAPve_g_L1_VR_1/1 -> IMAPve_g_L1_VR_2/1
  IMAPve_d_L1_Q/1 -> IMAPve_d_L1_Q_1/1
  IMAPve_d_L1_Q_1/1 -> IMAPve_d_L1_Q_2/1
  IMAPve_d_L1_Type/1 -> IMAPve_d_L1_Type_1/1
  IMAPve_d_L1_Type_1/1 -> IMAPve_d_L1_Type_2/1
  IMAPve_g_L1_Confidence/1 -> IMAPve_g_L1_Confidence_1/1
  IMAPve_g_L1_Confidence_1/1 -> IMAPve_g_L1_Confidence_2/1
  IMAPve_g_L1_W/1 -> IMAPve_g_L1_W_1/1
  IMAPve_g_L1_W_1/1 -> IMAPve_g_L1_W_2/1
  IMAPve_g_L1_TLC/1 -> IMAPve_g_L1_TLC_1/1
  IMAPve_g_L1_TLC_1/1 -> IMAPve_g_L1_TLC_2/1
  IMAPve_d_L1_LC/1 -> IMAPve_d_L1_LC_1/1
  IMAPve_d_L1_LC_1/1 -> IMAPve_d_L1_LC_2/1
  IMAPve_g_R1_C0/1 -> IMAPve_g_R1_C0_1/1
  IMAPve_g_R1_C0_1/1 -> IMAPve_g_R1_C0_2/1
  IMAPve_g_R1_C1/1 -> IMAPve_g_R1_C1_1/1
  IMAPve_g_R1_C1_1/1 -> IMAPve_g_R1_C1_2/1
  IMAPve_g_R1_C2/1 -> IMAPve_g_R1_C2_1/1
  IMAPve_g_R1_C2_1/1 -> IMAPve_g_R1_C2_2/1
  IMAPve_g_R1_C3/1 -> IMAPve_g_R1_C3_1/1
  IMAPve_g_R1_C3_1/1 -> IMAPve_g_R1_C3_2/1
  IMAPve_g_R1_VR/1 -> IMAPve_g_R1_VR_1/1
  IMAPve_g_R1_VR_1/1 -> IMAPve_g_R1_VR_2/1
  IMAPve_d_R1_Q/1 -> IMAPve_d_R1_Q_1/1
  IMAPve_d_R1_Q_1/1 -> IMAPve_d_R1_Q_2/1
  IMAPve_d_R1_Type/1 -> IMAPve_d_R1_Type_1/1
  IMAPve_d_R1_Type_1/1 -> IMAPve_d_R1_Type_2/1
  IMAPve_g_R1_Confidence/1 -> IMAPve_g_R1_Confidence_1/1
  IMAPve_g_R1_Confidence_1/1 -> IMAPve_g_R1_Confidence_2/1
  IMAPve_g_R1_W/1 -> IMAPve_g_R1_W_1/1
  IMAPve_g_R1_W_1/1 -> IMAPve_g_R1_W_2/1
  IMAPve_g_R1_TLC/1 -> IMAPve_g_R1_TLC_1/1
  IMAPve_g_R1_TLC_1/1 -> IMAPve_g_R1_TLC_2/1
  IMAPve_d_R1_LC/1 -> IMAPve_d_R1_LC_1/1
  IMAPve_d_R1_LC_1/1 -> IMAPve_d_R1_LC_2/1
  IMAPve_g_L0_C0_Back/1 -> IMAPve_g_L0_C0_Back_1/1
  IMAPve_g_L0_C0_Back_1/1 -> IMAPve_g_L0_C0_Back_2/1
  IMAPve_g_L0_C1_Back/1 -> IMAPve_g_L0_C1_Back_1/1
  IMAPve_g_L0_C1_Back_1/1 -> IMAPve_g_L0_C1_Back_2/1
  IMAPve_g_L0_C2_Back/1 -> IMAPve_g_L0_C2_Back_1/1
  IMAPve_g_L0_C2_Back_1/1 -> IMAPve_g_L0_C2_Back_2/1
  IMAPve_g_L0_C3_Back/1 -> IMAPve_g_L0_C3_Back_1/1
  IMAPve_g_L0_C3_Back_1/1 -> IMAPve_g_L0_C3_Back_2/1
  IMAPve_g_L0_Range_Back/1 -> IMAPve_g_L0_Range_Back_1/1
  IMAPve_g_L0_Range_Back_1/1 -> IMAPve_g_L0_Range_Back_2/1
  IMAPve_g_L0_C0_FR_Pred/1 -> IMAPve_g_L0_C0_FR_Pred_1/1
  IMAPve_g_L0_C0_FR_Pred_1/1 -> IMAPve_g_L0_C0_FR_Pred_2/1
  IMAPve_g_L0_C1_FR_Pred/1 -> IMAPve_g_L0_C1_FR_Pred_1/1
  IMAPve_g_L0_C1_FR_Pred_1/1 -> IMAPve_g_L0_C1_FR_Pred_2/1
  IMAPve_g_L0_C2_FR_Pred/1 -> IMAPve_g_L0_C2_FR_Pred_1/1
  IMAPve_g_L0_C2_FR_Pred_1/1 -> IMAPve_g_L0_C2_FR_Pred_2/1
  IMAPve_g_L0_Range_FR_Pred/1 -> IMAPve_g_L0_Range_FR_Pred_1/1
  IMAPve_g_L0_Range_FR_Pred_1/1 -> IMAPve_g_L0_Range_FR_Pred_2/1
  IMAPve_g_R0_C0_Back/1 -> IMAPve_g_R0_C0_Back_1/1
  IMAPve_g_R0_C0_Back_1/1 -> IMAPve_g_R0_C0_Back_2/1
  IMAPve_g_R0_C1_Back/1 -> IMAPve_g_R0_C1_Back_1/1
  IMAPve_g_R0_C1_Back_1/1 -> IMAPve_g_R0_C1_Back_2/1
  IMAPve_g_R0_C2_Back/1 -> IMAPve_g_R0_C2_Back_1/1
  IMAPve_g_R0_C2_Back_1/1 -> IMAPve_g_R0_C2_Back_2/1
  IMAPve_g_R0_C3_Back/1 -> IMAPve_g_R0_C3_Back_1/1
  IMAPve_g_R0_C3_Back_1/1 -> IMAPve_g_R0_C3_Back_2/1
  IMAPve_g_R0_Range_Back/1 -> IMAPve_g_R0_Range_Back_1/1
  IMAPve_g_R0_Range_Back_1/1 -> IMAPve_g_R0_Range_Back_2/1
  IMAPve_g_R0_C0_FR_Pred/1 -> IMAPve_g_R0_C0_FR_Pred_1/1
  IMAPve_g_R0_C0_FR_Pred_1/1 -> IMAPve_g_R0_C0_FR_Pred_2/1
  IMAPve_g_R0_C1_FR_Pred/1 -> IMAPve_g_R0_C1_FR_Pred_1/1
  IMAPve_g_R0_C1_FR_Pred_1/1 -> IMAPve_g_R0_C1_FR_Pred_2/1
  IMAPve_g_R0_C2_FR_Pred/1 -> IMAPve_g_R0_C2_FR_Pred_1/1
  IMAPve_g_R0_C2_FR_Pred_1/1 -> IMAPve_g_R0_C2_FR_Pred_2/1
  IMAPve_g_R0_Range_FR_Pred/1 -> IMAPve_g_R0_Range_FR_Pred_1/1
  IMAPve_g_R0_Range_FR_Pred_1/1 -> IMAPve_g_R0_Range_FR_Pred_2/1
  IMAPve_g_L1_C0_Back/1 -> IMAPve_g_L1_C0_Back_1/1
  IMAPve_g_L1_C0_Back_1/1 -> IMAPve_g_L1_C0_Back_2/1
  IMAPve_g_L1_C1_Back/1 -> IMAPve_g_L1_C1_Back_1/1
  IMAPve_g_L1_C1_Back_1/1 -> IMAPve_g_L1_C1_Back_2/1
  IMAPve_g_L1_C2_Back/1 -> IMAPve_g_L1_C2_Back_1/1
  IMAPve_g_L1_C2_Back_1/1 -> IMAPve_g_L1_C2_Back_2/1
  IMAPve_g_L1_C3_Back/1 -> IMAPve_g_L1_C3_Back_1/1
  IMAPve_g_L1_C3_Back_1/1 -> IMAPve_g_L1_C3_Back_2/1
  IMAPve_g_L1_Range_Back/1 -> IMAPve_g_L1_Range_Back_1/1
  IMAPve_g_L1_Range_Back_1/1 -> IMAPve_g_L1_Range_Back_2/1
  IMAPve_g_L1_C0_FR_Pred/1 -> IMAPve_g_L1_C0_FR_Pred_1/1
  IMAPve_g_L1_C0_FR_Pred_1/1 -> IMAPve_g_L1_C0_FR_Pred_2/1
  IMAPve_g_L1_C1_FR_Pred/1 -> IMAPve_g_L1_C1_FR_Pred_1/1
  IMAPve_g_L1_C1_FR_Pred_1/1 -> IMAPve_g_L1_C1_FR_Pred_2/1
  IMAPve_g_L1_C2_FR_Pred/1 -> IMAPve_g_L1_C2_FR_Pred_1/1
  IMAPve_g_L1_C2_FR_Pred_1/1 -> IMAPve_g_L1_C2_FR_Pred_2/1
  IMAPve_g_L1_Range_FR_Pred/1 -> IMAPve_g_L1_Range_FR_Pred_1/1
  IMAPve_g_L1_Range_FR_Pred_1/1 -> IMAPve_g_L1_Range_FR_Pred_2/1
  IMAPve_g_R1_C0_Back/1 -> IMAPve_g_R1_C0_Back_1/1
  IMAPve_g_R1_C0_Back_1/1 -> IMAPve_g_R1_C0_Back_2/1
  IMAPve_g_R1_C1_Back/1 -> IMAPve_g_R1_C1_Back_1/1
  IMAPve_g_R1_C1_Back_1/1 -> IMAPve_g_R1_C1_Back_2/1
  IMAPve_g_R1_C2_Back/1 -> IMAPve_g_R1_C2_Back_1/1
  IMAPve_g_R1_C2_Back_1/1 -> IMAPve_g_R1_C2_Back_2/1
  IMAPve_g_R1_C3_Back/1 -> IMAPve_g_R1_C3_Back_1/1
  IMAPve_g_R1_C3_Back_1/1 -> IMAPve_g_R1_C3_Back_2/1
  IMAPve_g_R1_Range_Back/1 -> IMAPve_g_R1_Range_Back_1/1
  IMAPve_g_R1_Range_Back_1/1 -> IMAPve_g_R1_Range_Back_2/1
  IMAPve_g_R1_C0_FR_Pred/1 -> IMAPve_g_R1_C0_FR_Pred_1/1
  IMAPve_g_R1_C0_FR_Pred_1/1 -> IMAPve_g_R1_C0_FR_Pred_2/1
  IMAPve_g_R1_C1_FR_Pred/1 -> IMAPve_g_R1_C1_FR_Pred_1/1
  IMAPve_g_R1_C1_FR_Pred_1/1 -> IMAPve_g_R1_C1_FR_Pred_2/1
  IMAPve_g_R1_C2_FR_Pred/1 -> IMAPve_g_R1_C2_FR_Pred_1/1
  IMAPve_g_R1_C2_FR_Pred_1/1 -> IMAPve_g_R1_C2_FR_Pred_2/1
  IMAPve_g_R1_Range_FR_Pred/1 -> IMAPve_g_R1_Range_FR_Pred_1/1
  IMAPve_g_R1_Range_FR_Pred_1/1 -> IMAPve_g_R1_Range_FR_Pred_2/1
  IMAPve_d_Sign_ISA_Value/1 -> IMAPve_d_Sign_ISA_Value_1/1
  IMAPve_d_Sign_ISA_Value_1/1 -> IMAPve_d_Sign_ISA_Value_2/1
  IMAPve_d_TSR_Sign_Type/1 -> IMAPve_d_TSR_Sign_Type_1/1
  IMAPve_d_TSR_Sign_Type_1/1 -> IMAPve_d_TSR_Sign_Type_2/1
  IMAPve_d_Camera_Signal_Fault/1 -> IMAPve_d_Camera_Signal_Fault_1/1
  IMAPve_d_Camera_Signal_Fault_1/1 -> IMAPve_d_Camera_Signal_Fault_2/1
  IMAPve_d_Radar_Status/1 -> IMAPve_d_Radar_Status_1/1
  IMAPve_d_Radar_Status_1/1 -> IMAPve_d_Radar_Status_2/1
  IMAPve_d_Camera_Status/1 -> IMAPve_d_Camera_Status_1/1
  IMAPve_d_Camera_Status_1/1 -> IMAPve_d_Camera_Status_2/1
  ICACve_g_SteerAngleCmd_1/1 -> ICACve_g_SteerAngleCmd/1
  ICACve_g_SteerAngleCmd_2/1 -> ICACve_g_SteerAngleCmd_1/1
  ICACve_d_SteerAngleVld_1/1 -> ICACve_d_SteerAngleVld/1
  ICACve_d_SteerAngleVld_2/1 -> ICACve_d_SteerAngleVld_1/1
  ICACve_d_SignalTStamp_1/1 -> ICACve_d_SignalTStamp/1
  ICACve_d_SignalTStamp_2/1 -> ICACve_d_SignalTStamp_1/1
